simulink model "IEEE_30_Bus_System_with_HVDC"  (R2021a)
settings: Solver=FixedStepDiscrete  StartTime=0.0  StopTime=15  FixedStep=Tss  RelTol=1e-3
InitFcn:
  | Tss=5e-5
  | 
  | Pnom = 20e6
  | Vdc = 40e3
  | 
  | Vbreak_on = Vdc + Vdc*150/800
  | Vbreak_off = Vdc
  | break_status_time = 1.0
  | 
  | Rbrk =  Vdc*Vdc/(1.0*Pnom)
  | 
  | Vg1rms = 33e3*1.0118
  | Lg1 = 20e-6
  | Rg1 = 10e-3
  | f1 = 60.0
  | m_f=27
  | fsw = 10000.0
  | Ilpp = 0.1*Pnom/Vg1rms
  | a = 10.0
  | 
  | ffast = 1.0*fsw
  | Tfast = 1.0/ffast
  | 
  | Rdc = Vdc*Vdc/Pnom
  | 
  | R1 = Vg1rms*Vg1rms / (500*Pnom) / 3.0
  | %L1 = 3.0*1.41*Vg1rms / (2*Vdc) * ((2.0/3.0*Vdc - 1.41*Vg1rms) / (Ilpp*fsw))
  | L1=8e-3
  | %Cf1 = (a+1)/(4*pi*pi*fsw*fsw*Lg1)
  | Cf1=4e-6
  | %C_dc = 100e-10*Pnom
  | C_dc=0.02
  | %R_dump = 1.0/(20.0*pi*f1*Cf1)*10000.0/Pnom
  | R_dump=20
  | 
  | p = -0.135*10.0
  | i = -0.004/2.0
  | 
  | Kp_i = 2*L1*fsw*p / Vdc / 2.0
  | Ki_i = 2*L1*fsw*i / Vdc / 2.0
  | 
  | Tsw = 1/fsw
  | 
  | Vg2rms = 33e3*1.0571
  | Lg2 = 20e-6
  | Rg2 = 10e-3
  | f2 = 60.0
  | fsw2 = 10000.0
  | Il2pp = 0.1*Pnom/Vg2rms
  | a2 = 10.0
  | 
  | R2 = Vg2rms*Vg2rms / (500*Pnom) / 3.0
  | %L2 = 3.0*1.41*Vg2rms / (2*Vdc) * ((2.0/3.0*Vdc - 1.41*Vg2rms) / (Il2pp*fsw2))
  | L2=20e-3
  | %Cf2 = (a2+1)/(4*pi*pi*fsw2*fsw2*Lg2)
  | Cf2=9e-6
  | 
  | %R_dump2 = 1.0/(20.0*pi*f2*Cf2)*10000.0/Pnom
  | R_dump2=20
  | 
  | Tsw2 = 1/fsw2
  | Tslow = 1e-3
  | 
  | p_v = 0.2403
  | i_v = 0.0549
  | 
  | Kp_v = 4*p_v / (1.5*Vg2rms*1.41*Tslow)
  | Ki_v = 4*i_v / (1.5*Vg2rms*1.41*Tslow)
  | 
  | Imax = Pnom/Vg2rms/3.0 * 1.41 * 2.0
undefined symbols (not defined in the file): Angle, DiscIntNeverNeededParam, Magnitude, V_890, Vnom1
libraries: spsThreePhasePISectionLineLib x37, spsThreePhaseVIMeasurementLib x32, spsLoadFlowBusLib x30, spsSeriesRLCBranchLib x27, spsThreePhaseSeriesRLCLoadLib x23, spsVoltageMeasurementLib x17, spsCurrentMeasurementLib x15, spsThreePhaseSourceLib x7, pid_lib x7, spsabctodq0Lib x6, spsFirstOrderFilterLib x4, eeGeneralControl x4
(part 1 of 2)
settings Model: SimulationMode=accelerator  Creator=liyifu  LastModifiedBy=l4729
settings SolverCC: AlgebraicLoopSolver=TrustRegion
settings DataIOCC: ReturnWorkspaceOutputs=off
settings DebuggingCC: UnconnectedInputMsg=none  UnconnectedOutputMsg=none  UnconnectedLineMsg=none  SFMachineParentedDataDiag=warning  ArithmeticOperatorsInVariantConditions=warning
settings SFSimCC: SimUseLocalCustomCode=off  CustomCodeUndefinedFunction=UseInterfaceOnly
settings RTWCC: RTWUseLocalCustomCode=off

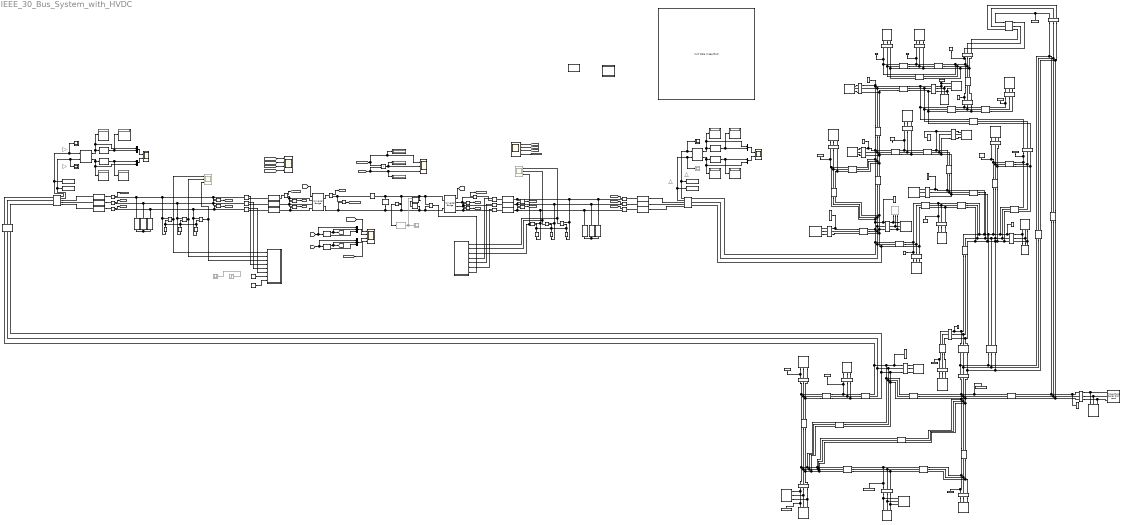
== system IEEE_30_Bus_System_with_HVDC ==
  note: IEEE 30 Node Test Feeder
  14 : spsThreePhaseVIMeasurementLib/Three-Phase V-I Measurement  VoltageMeasurement=phase-to-ground  SetLabelV=on  LabelV=Vabc_14  Vpu=on  VpuLL=off  CurrentMeasurement=yes  SetLabelI=on  LabelI=Iabc_14  Ipu=on  Pbase=100e6  Vbase=33e3  OutputType=Magnitude-Angle  PhasorSimulation=off  PSBequivalent=0
  15 : spsThreePhaseVIMeasurementLib/Three-Phase V-I Measurement  VoltageMeasurement=phase-to-ground  SetLabelV=on  LabelV=Vabc_15  Vpu=on  VpuLL=off  CurrentMeasurement=yes  SetLabelI=on  LabelI=Iabc_15  Ipu=on  Pbase=100e6  Vbase=33e3  OutputType=Magnitude-Angle  PhasorSimulation=off  PSBequivalent=0
  16 : spsThreePhaseVIMeasurementLib/Three-Phase V-I Measurement  VoltageMeasurement=phase-to-ground  SetLabelV=on  LabelV=Vabc_16  Vpu=on  VpuLL=off  CurrentMeasurement=yes  SetLabelI=on  LabelI=Iabc_16  Ipu=on  Pbase=100e6  Vbase=33e3  OutputType=Magnitude-Angle  PhasorSimulation=off  PSBequivalent=0
  17 : spsThreePhaseVIMeasurementLib/Three-Phase V-I Measurement  VoltageMeasurement=phase-to-ground  SetLabelV=on  LabelV=Vabc_17  Vpu=on  VpuLL=off  CurrentMeasurement=yes  SetLabelI=on  LabelI=Iabc_17  Ipu=on  Pbase=100e6  Vbase=33e3  OutputType=Magnitude-Angle  PhasorSimulation=off  PSBequivalent=0
  18 : spsThreePhaseVIMeasurementLib/Three-Phase V-I Measurement  VoltageMeasurement=phase-to-ground  SetLabelV=on  LabelV=Vabc_18  Vpu=on  VpuLL=off  CurrentMeasurement=yes  SetLabelI=on  LabelI=Iabc_18  Ipu=on  Pbase=100e6  Vbase=33e3  OutputType=Magnitude-Angle  PhasorSimulation=off  PSBequivalent=0
  19 : spsThreePhaseVIMeasurementLib/Three-Phase V-I Measurement  VoltageMeasurement=phase-to-ground  SetLabelV=on  LabelV=Vabc_19  Vpu=on  VpuLL=off  CurrentMeasurement=yes  SetLabelI=on  LabelI=Iabc_19  Ipu=on  Pbase=100e6  Vbase=33e3  OutputType=Magnitude-Angle  PhasorSimulation=off  PSBequivalent=0
  20 : spsThreePhaseVIMeasurementLib/Three-Phase V-I Measurement  VoltageMeasurement=phase-to-ground  SetLabelV=on  LabelV=Vabc_20  Vpu=on  VpuLL=off  CurrentMeasurement=yes  SetLabelI=on  LabelI=Iabc_20  Ipu=on  Pbase=100e6  Vbase=33e3  OutputType=Magnitude-Angle  PhasorSimulation=off  PSBequivalent=0
  21 : spsThreePhaseVIMeasurementLib/Three-Phase V-I Measurement  VoltageMeasurement=phase-to-ground  SetLabelV=on  LabelV=Vabc_21  Vpu=on  VpuLL=off  CurrentMeasurement=yes  SetLabelI=on  LabelI=Iabc_21  Ipu=on  Pbase=100e6  Vbase=33e3  OutputType=Magnitude-Angle  PhasorSimulation=off  PSBequivalent=0
  22 : spsThreePhaseVIMeasurementLib/Three-Phase V-I Measurement  VoltageMeasurement=phase-to-ground  SetLabelV=on  LabelV=Vabc_22  Vpu=on  VpuLL=off  CurrentMeasurement=yes  SetLabelI=on  LabelI=Iabc_22  Ipu=on  Pbase=100e6  Vbase=33e3  OutputType=Magnitude-Angle  PhasorSimulation=off  PSBequivalent=0
  23 : spsThreePhaseVIMeasurementLib/Three-Phase V-I Measurement  VoltageMeasurement=phase-to-ground  SetLabelV=on  LabelV=Vabc_23  Vpu=on  VpuLL=off  CurrentMeasurement=yes  SetLabelI=on  LabelI=Iabc_23  Ipu=on  Pbase=100e6  Vbase=33e3  OutputType=Magnitude-Angle  PhasorSimulation=off  PSBequivalent=0
  24 : spsThreePhaseVIMeasurementLib/Three-Phase V-I Measurement  VoltageMeasurement=phase-to-ground  SetLabelV=on  LabelV=Vabc_24  Vpu=on  VpuLL=off  CurrentMeasurement=yes  SetLabelI=on  LabelI=Iabc_24  Ipu=on  Pbase=100e6  Vbase=33e3  OutputType=Magnitude-Angle  PhasorSimulation=off  PSBequivalent=0
  25 : spsThreePhaseVIMeasurementLib/Three-Phase V-I Measurement  VoltageMeasurement=phase-to-ground  SetLabelV=on  LabelV=Vabc_25  Vpu=on  VpuLL=off  CurrentMeasurement=yes  SetLabelI=on  LabelI=Iabc_25  Ipu=on  Pbase=100e6  Vbase=33e3  OutputType=Magnitude-Angle  PhasorSimulation=off  PSBequivalent=0
  26 : spsThreePhaseVIMeasurementLib/Three-Phase V-I Measurement  VoltageMeasurement=phase-to-ground  SetLabelV=on  LabelV=Vabc_26  Vpu=on  VpuLL=off  CurrentMeasurement=yes  SetLabelI=on  LabelI=Iabc_26  Ipu=on  Pbase=100e6  Vbase=33e3  OutputType=Magnitude-Angle  PhasorSimulation=off  PSBequivalent=0
  29 : spsThreePhaseVIMeasurementLib/Three-Phase V-I Measurement  VoltageMeasurement=phase-to-ground  SetLabelV=on  LabelV=Vabc_29  Vpu=on  VpuLL=off  CurrentMeasurement=yes  SetLabelI=on  LabelI=Iabc_29  Ipu=on  Pbase=100e6  Vbase=33e3  OutputType=Magnitude-Angle  PhasorSimulation=off  PSBequivalent=0
  30 : spsThreePhaseVIMeasurementLib/Three-Phase V-I Measurement  VoltageMeasurement=phase-to-ground  SetLabelV=on  LabelV=Vabc_30  Vpu=on  VpuLL=off  CurrentMeasurement=yes  SetLabelI=on  LabelI=Iabc_30  Ipu=on  Pbase=100e6  Vbase=33e3  OutputType=Magnitude-Angle  PhasorSimulation=off  PSBequivalent=0
  Blaine : spsThreePhaseVIMeasurementLib/Three-Phase V-I Measurement  VoltageMeasurement=phase-to-ground  SetLabelV=on  LabelV=Vabc_7  Vpu=on  VpuLL=off  CurrentMeasurement=yes  SetLabelI=on  LabelI=Iabc_7  Ipu=on  Pbase=100e6  Vbase=132e3  OutputType=Magnitude-Angle  PhasorSimulation=off  PSBequivalent=0
  Break control1 : Subsystem  Commented=on
  Breaker1 : spsBreakerLib/Breaker  InitialState=0  SwitchingTimes="[1/60  5/60]"  External=on  BreakerResistance=0.01  SnubberResistance=1e6  SnubberCapacitance=inf  Measurements=None  MoreParameters=on  NoBreakLoop=off
      settings: SourceProductBaseCode=PS
  Claytor : spsThreePhaseVIMeasurementLib/Three-Phase V-I Measurement  VoltageMeasurement=phase-to-ground  SetLabelV=on  LabelV=Vabc_2  Vpu=on  VpuLL=off  CurrentMeasurement=yes  SetLabelI=on  LabelI=Iabc_2  Ipu=on  Pbase=100e6  Vbase=132e3  OutputType=Magnitude-Angle  PhasorSimulation=off  PSBequivalent=0
  Cloverdl : spsThreePhaseVIMeasurementLib/Three-Phase V-I Measurement  VoltageMeasurement=phase-to-ground  SetLabelV=on  LabelV=Vabc_27  Vpu=on  VpuLL=off  CurrentMeasurement=yes  SetLabelI=on  LabelI=Iabc_27  Ipu=on  Pbase=100e6  Vbase=33e3  OutputType=Magnitude-Angle  PhasorSimulation=off  PSBequivalent=0
  Cloverdl1 : spsThreePhaseVIMeasurementLib/Three-Phase V-I Measurement  VoltageMeasurement=phase-to-ground  SetLabelV=on  LabelV=Vabc_28  Vpu=on  VpuLL=off  CurrentMeasurement=yes  SetLabelI=on  LabelI=Iabc_28  Ipu=on  Pbase=100e6  Vbase=132e3  OutputType=Magnitude-Angle  PhasorSimulation=off  PSBequivalent=0
  Constant3 : Constant  Value=5e6
  Constant4 : Constant  Value=1e6
  Current Measurement{1..15} (15 alike) : spsCurrentMeasurementLib/Current Measurement  PhasorSimulation=off  OutputType=Complex  PSBequivalent=0
  Display{1..2,6..8,13..18} (11 alike) : Display
  Equivalent Gen : spsThreePhaseSourceLib/Three-Phase Source  Commented=on  InternalConnection=Yg  VoltagePhases=off  Voltage=(33000)*1.04012  PhaseAngle=92.4376  Voltage_phases=[33 33 33]*1e3/sqrt(3)  PhaseAngles_phases=[0 -120 +120]  Frequency=60  NonIdealSource=on  SpecifyImpedance=off  Resistance=10  Inductance=0.15  ShortCircuitLevel=Apparent_power_gen1  BaseVoltage=33e3  XRratio=8  BusType=PQ  Pref=1000000  Qref=0  Prefabc=[10e3, 10e3, 10e3]  Qrefabc=[0, 0, 0]  Qmin=-Inf  Qmax=Inf
  Fieldale : spsThreePhaseVIMeasurementLib/Three-Phase V-I Measurement  VoltageMeasurement=phase-to-ground  SetLabelV=on  LabelV=Vabc_5  Vpu=on  VpuLL=off  CurrentMeasurement=yes  SetLabelI=on  LabelI=Iabc_5  Ipu=on  Pbase=100e6  Vbase=132e3  OutputType=Magnitude-Angle  PhasorSimulation=off  PSBequivalent=0
  Gain4 : Gain  Commented=on  Gain=33e3*sqrt(2)/sqrt(3)
  Gain5 : Gain  Commented=on  Gain=100e6/33e3*sqrt(2)/sqrt(3)
  Gain6 : Gain  Commented=on  Gain=33e3*sqrt(2)/sqrt(3)
  Gain7 : Gain  Commented=on  Gain=100e6/33e3*sqrt(2)/sqrt(3)
  Gen1 : spsThreePhaseSourceLib/Three-Phase Source  InternalConnection=Yg  VoltagePhases=off  Voltage=(132000)*1.37988  PhaseAngle=133.6021  Voltage_phases=[132 132 132]*1e3/sqrt(3)  PhaseAngles_phases=[0 -120 +120]  Frequency=60  NonIdealSource=on  SpecifyImpedance=off  Resistance=10  Inductance=0.15  ShortCircuitLevel=Apparent_power_gen1  BaseVoltage=132e3  XRratio=8  BusType=swing  Pref=2.6095  Qref=-0.1679  Prefabc=[10e3, 10e3, 10e3]  Qrefabc=[0, 0, 0]  Qmin=-Inf  Qmax=Inf
  Gen2 : spsThreePhaseSourceLib/Three-Phase Source  InternalConnection=Yg  VoltagePhases=off  Voltage=(132000)*1.17992  PhaseAngle=98.3264  Voltage_phases=[132 132 132]*1e3/sqrt(3)  PhaseAngles_phases=[0 -120 +120]  Frequency=60  NonIdealSource=on  SpecifyImpedance=off  Resistance=10  Inductance=0.15  ShortCircuitLevel=Apparent_power_gen1  BaseVoltage=132e3  XRratio=8  BusType=PV  Pref=40000000  Qref=0.5  Prefabc=[10e3, 10e3, 10e3]  Qrefabc=[0, 0, 0]  Qmin=-Inf  Qmax=Inf
  Gen3 : spsThreePhaseSourceLib/Three-Phase Source  InternalConnection=Yg  VoltagePhases=off  Voltage=(132000)*1.11434  PhaseAngle=83.6097  Voltage_phases=[132 132 132]*1e3/sqrt(3)  PhaseAngles_phases=[0 -120 +120]  Frequency=60  NonIdealSource=on  SpecifyImpedance=off  Resistance=10  Inductance=0.15  ShortCircuitLevel=Apparent_power_gen1  BaseVoltage=132e3  XRratio=8  BusType=PV  Pref=0  Qref=0.3685  Prefabc=[10e3, 10e3, 10e3]  Qrefabc=[0, 0, 0]  Qmin=-Inf  Qmax=Inf
  Gen4 : spsThreePhaseSourceLib/Three-Phase Source  InternalConnection=Yg  VoltagePhases=off  Voltage=(132000)*1.0549  PhaseAngle=86.5606  Voltage_phases=[132 132 132]*1e3/sqrt(3)  PhaseAngles_phases=[0 -120 +120]  Frequency=60  NonIdealSource=on  SpecifyImpedance=off  Resistance=10  Inductance=0.15  ShortCircuitLevel=Apparent_power_gen1  BaseVoltage=132e3  XRratio=8  BusType=PV  Pref=0  Qref=0.3714  Prefabc=[10e3, 10e3, 10e3]  Qrefabc=[0, 0, 0]  Qmin=-Inf  Qmax=Inf
  Gen5 : spsThreePhaseSourceLib/Three-Phase Source  InternalConnection=Yg  VoltagePhases=off  Voltage=(33000)*2.66924  PhaseAngle=81.613  Voltage_phases=[33 33 33]*1e3/sqrt(3)  PhaseAngles_phases=[0 -120 +120]  Frequency=60  NonIdealSource=on  SpecifyImpedance=off  Resistance=10  Inductance=0.15  ShortCircuitLevel=Apparent_power_gen1  BaseVoltage=33e3  XRratio=8  BusType=PV  Pref=0  Qref=0.1617  Prefabc=[10e3, 10e3, 10e3]  Qrefabc=[0, 0, 0]  Qmin=-Inf  Qmax=Inf
  Gen6 : spsThreePhaseSourceLib/Three-Phase Source  InternalConnection=Yg  VoltagePhases=off  Voltage=(33000)*2.72717  PhaseAngle=83.0417  Voltage_phases=[33 33 33]*1e3/sqrt(3)  PhaseAngles_phases=[0 -120 +120]  Frequency=60  NonIdealSource=on  SpecifyImpedance=off  Resistance=10  Inductance=0.15  ShortCircuitLevel=Apparent_power_gen1  BaseVoltage=33e3  XRratio=8  BusType=PV  Pref=0  Qref=0.1062  Prefabc=[10e3, 10e3, 10e3]  Qrefabc=[0, 0, 0]  Qmin=-Inf  Qmax=Inf
  Glen Lyn : spsThreePhaseVIMeasurementLib/Three-Phase V-I Measurement  VoltageMeasurement=phase-to-ground  SetLabelV=on  LabelV=Vabc_1  Vpu=on  VpuLL=off  CurrentMeasurement=yes  SetLabelI=on  LabelI=Iabc_1  Ipu=on  Pbase=100e6  Vbase=132e3  OutputType=Magnitude-Angle  PhasorSimulation=off  PSBequivalent=0
  Hancock : spsThreePhaseVIMeasurementLib/Three-Phase V-I Measurement  VoltageMeasurement=phase-to-ground  SetLabelV=on  LabelV=Vabc_4  Vpu=on  VpuLL=off  CurrentMeasurement=yes  SetLabelI=on  LabelI=Iabc_4  Ipu=on  Pbase=100e6  Vbase=132e3  OutputType=Magnitude-Angle  PhasorSimulation=off  PSBequivalent=0
  Hancock1 : spsThreePhaseVIMeasurementLib/Three-Phase V-I Measurement  VoltageMeasurement=phase-to-ground  SetLabelV=on  LabelV=Vabc_12  Vpu=on  VpuLL=off  CurrentMeasurement=yes  SetLabelI=on  LabelI=Iabc_12  Ipu=on  Pbase=100e6  Vbase=33e3  OutputType=Magnitude-Angle  PhasorSimulation=off  PSBequivalent=0
  Hancock2 : spsThreePhaseVIMeasurementLib/Three-Phase V-I Measurement  VoltageMeasurement=phase-to-ground  SetLabelV=on  LabelV=Vabc_13  Vpu=on  VpuLL=off  CurrentMeasurement=yes  SetLabelI=on  LabelI=Iabc_13  Ipu=on  Pbase=100e6  Vbase=33e3  OutputType=Magnitude-Angle  PhasorSimulation=off  PSBequivalent=0
  Inverter Control : Subsystem
  Kumis : spsThreePhaseVIMeasurementLib/Three-Phase V-I Measurement  VoltageMeasurement=phase-to-ground  SetLabelV=on  LabelV=Vabc_3  Vpu=on  VpuLL=off  CurrentMeasurement=yes  SetLabelI=on  LabelI=Iabc_3  Ipu=on  Pbase=100e6  Vbase=132e3  OutputType=Magnitude-Angle  PhasorSimulation=off  PSBequivalent=0
  L1-2 : spsThreePhasePISectionLineLib/Three-Phase PI Section Line  LConnTagsString=a|b|c  RConnTagsString=A|B|C  Length=1  Frequency=60  Resistances=[0.0192 0.048]*174.24  Inductances=[1.5252e-4 3.8131e-4]*174.24  Capacitances=[1.4006e-4 1.4006e-4]/174.24
  L1-3 : spsThreePhasePISectionLineLib/Three-Phase PI Section Line  LConnTagsString=a|b|c  RConnTagsString=A|B|C  Length=1  Frequency=60  Resistances=[0.0452 0.113]*174.24  Inductances=[4.3821e-4 1.0955e-4]*174.24  Capacitances=[1.0823e-4 1.0823e-4]/174.24
  L10-17 : spsThreePhasePISectionLineLib/Three-Phase PI Section Line  LConnTagsString=a|b|c  RConnTagsString=A|B|C  Length=1  Frequency=60  Resistances=[0.0324 0.081]*10.89  Inductances=[2.2414e-4 5.6036e-4]*10.89  Capacitances=[1e-6 1e-6]/10.89
  L10-20 : spsThreePhasePISectionLineLib/Three-Phase PI Section Line  LConnTagsString=a|b|c  RConnTagsString=A|B|C  Length=1  Frequency=60  Resistances=[0.0936 0.234]*10.89  Inductances=[5.5439e-4 1.3860e-3]*10.89  Capacitances=[1e-6 1e-6]/10.89
  L10-21 : spsThreePhasePISectionLineLib/Three-Phase PI Section Line  LConnTagsString=a|b|c  RConnTagsString=A|B|C  Length=1  Frequency=60  Resistances=[0.0348 0.087]*10.89  Inductances=[1.9868e-4 4.9670e-4]*10.89  Capacitances=[1e-6 1e-6]/10.89
  L10-22 : spsThreePhasePISectionLineLib/Three-Phase PI Section Line  LConnTagsString=a|b|c  RConnTagsString=A|B|C  Length=1  Frequency=60  Resistances=[0.0727 0.18175]*10.89  Inductances=[3.9762e-4 9.9406e-4]*10.89  Capacitances=[1e-6 1e-6]/10.89
  L12-13 : spsThreePhasePISectionLineLib/Three-Phase PI Section Line  LConnTagsString=a|b|c  RConnTagsString=A|B|C  Length=1  Frequency=60  Resistances=[0 0]*10.89  Inductances=[3.7136e-4 9.2840e-4]*10.89  Capacitances=[1e-6 1e-6]/10.89
  L12-14 : spsThreePhasePISectionLineLib/Three-Phase PI Section Line  LConnTagsString=a|b|c  RConnTagsString=A|B|C  Length=1  Frequency=60  Resistances=[0.1231 0.30775]*10.89  Inductances=[6.7880e-4 1.6970e-3]*10.89  Capacitances=[1e-6 1e-6]/10.89
  L12-15 : spsThreePhasePISectionLineLib/Three-Phase PI Section Line  LConnTagsString=a|b|c  RConnTagsString=A|B|C  Length=1  Frequency=60  Resistances=[0.0662 0.1655]*10.89  Inductances=[3.4590e-4 8.6474e-4]*10.89  Capacitances=[1e-6 1e-6]/10.89
  L12-16 : spsThreePhasePISectionLineLib/Three-Phase PI Section Line  LConnTagsString=a|b|c  RConnTagsString=A|B|C  Length=1  Frequency=60  Resistances=[0.0945 0.23625]*10.89  Inductances=[5.2707e-4 1.3177e-3]*10.89  Capacitances=[1e-6 1e-6]/10.89
  L14-15 : spsThreePhasePISectionLineLib/Three-Phase PI Section Line  LConnTagsString=a|b|c  RConnTagsString=A|B|C  Length=1  Frequency=60  Resistances=[0.221 0.5525]*10.89  Inductances=[5.2972e-4 1.3243e-3]*10.89  Capacitances=[1e-6 1e-6]/10.89
  L15-18 : spsThreePhasePISectionLineLib/Three-Phase PI Section Line  LConnTagsString=a|b|c  RConnTagsString=A|B|C  Length=1  Frequency=60  Resistances=[0.1073 0.26825]*10.89  Inductances=[5.7959e-4 1.4490e-3]*10.89  Capacitances=[1e-6 1e-6]/10.89
  L15-23 : spsThreePhasePISectionLineLib/Three-Phase PI Section Line  LConnTagsString=a|b|c  RConnTagsString=A|B|C  Length=1  Frequency=60  Resistances=[0.1 0.25]*10.89  Inductances=[5.3582e-4 1.3396e-3]*10.89  Capacitances=[1e-6 1e-6]/10.89
  L16-17 : spsThreePhasePISectionLineLib/Three-Phase PI Section Line  LConnTagsString=a|b|c  RConnTagsString=A|B|C  Length=1  Frequency=60  Resistances=[0.0524 0.131]*10.89  Inductances=[5.1009e-4 1.2752e-3]*10.89  Capacitances=[1e-6 1e-6]/10.89
  L18-19 : spsThreePhasePISectionLineLib/Three-Phase PI Section Line  LConnTagsString=a|b|c  RConnTagsString=A|B|C  Length=1  Frequency=60  Resistances=[0.0639 0.15975]*10.89  Inductances=[3.4271e-4 8.5678e-4]*10.89  Capacitances=[1e-6 1e-6]/10.89
  L19-20 : spsThreePhasePISectionLineLib/Three-Phase PI Section Line  LConnTagsString=a|b|c  RConnTagsString=A|B|C  Length=1  Frequency=60  Resistances=[0.034 0.085]*10.89  Inductances=[1.8038e-4 4.5094e-4]*10.89  Capacitances=[1e-6 1e-6]/10.89
  L2-4 : spsThreePhasePISectionLineLib/Three-Phase PI Section Line  LConnTagsString=a|b|c  RConnTagsString=A|B|C  Length=1  Frequency=60  Resistances=[0.057 0.1425]*174.24  Inductances=[4.6075e-4 1.1519e-3]*174.24  Capacitances=[9.7615e-5 9.7615e-5]/174.24
  L2-5 : spsThreePhasePISectionLineLib/Three-Phase PI Section Line  LConnTagsString=a|b|c  RConnTagsString=A|B|C  Length=1  Frequency=60  Resistances=[0.0472 0.118]*174.24  Inductances=[5.2601e-4 1.3150e-3]*174.24  Capacitances=[1.1088e-4 1.1088e-4]/174.24
  L2-6 : spsThreePhasePISectionLineLib/Three-Phase PI Section Line  LConnTagsString=a|b|c  RConnTagsString=A|B|C  Length=1  Frequency=60  Resistances=[0.0581 0.14525]*174.24  Inductances=[4.6765e-4 1.1691e-3]*174.24  Capacitances=[9.9206e-5 9.9206e-5]/174.24
  L21-22 : spsThreePhasePISectionLineLib/Three-Phase PI Section Line  LConnTagsString=a|b|c  RConnTagsString=A|B|C  Length=1  Frequency=60  Resistances=[0.0116 0.029]*10.89  Inductances=[6.2601e-5 1.5650e-4]*10.89  Capacitances=[1e-6 1e-6]/10.89
  L22-24 : spsThreePhasePISectionLineLib/Three-Phase PI Section Line  LConnTagsString=a|b|c  RConnTagsString=A|B|C  Length=1  Frequency=60  Resistances=[0.115 0.2875]*10.89  Inductances=[4.7481e-4 1.1870e-3]*10.89  Capacitances=[1e-6 1e-6]/10.89
  L23-24 : spsThreePhasePISectionLineLib/Three-Phase PI Section Line  LConnTagsString=a|b|c  RConnTagsString=A|B|C  Length=1  Frequency=60  Resistances=[0.132 0.33]*10.89  Inductances=[7.1620e-4 1.7905e-3]*10.89  Capacitances=[1e-6 1e-6]/10.89
  L24-25 : spsThreePhasePISectionLineLib/Three-Phase PI Section Line  LConnTagsString=a|b|c  RConnTagsString=A|B|C  Length=1  Frequency=60  Resistances=[0.1885 0.47125]*10.89  Inductances=[8.7323e-4 2.1831e-3]*10.89  Capacitances=[1e-6 1e-6]/10.89
  L25-26 : spsThreePhasePISectionLineLib/Three-Phase PI Section Line  LConnTagsString=a|b|c  RConnTagsString=A|B|C  Length=1  Frequency=60  Resistances=[0.2544 0.636]*10.89  Inductances=[1.008e-3 2.5200e-3]*10.89  Capacitances=[1e-6 1e-6]/10.89
  L25-27 : spsThreePhasePISectionLineLib/Three-Phase PI Section Line  LConnTagsString=a|b|c  RConnTagsString=A|B|C  Length=1  Frequency=60  Resistances=[0.1093 0.27325]*10.89  Inductances=[5.5360e-4 1.3840e-3]*10.89  Capacitances=[1e-6 1e-6]/10.89
  L27-29 : spsThreePhasePISectionLineLib/Three-Phase PI Section Line  LConnTagsString=a|b|c  RConnTagsString=A|B|C  Length=1  Frequency=60  Resistances=[0.2198 0.5495]*10.89  Inductances=[1.1016e-3 2.7540e-3]*10.89  Capacitances=[1e-6 1e-6]/10.89
  L27-30 : spsThreePhasePISectionLineLib/Three-Phase PI Section Line  LConnTagsString=a|b|c  RConnTagsString=A|B|C  Length=1  Frequency=60  Resistances=[0.3202 0.8005]*10.89  Inductances=[1.5987e-3 3.9968e-3]*10.89  Capacitances=[1e-6 1e-6]/10.89
  L29-30 : spsThreePhasePISectionLineLib/Three-Phase PI Section Line  LConnTagsString=a|b|c  RConnTagsString=A|B|C  Length=1  Frequency=60  Resistances=[0.2399 0.59975]*10.89  Inductances=[1.2024e-3 3.0060e-3]*10.89  Capacitances=[1e-6 1e-6]/10.89
  L3-4 : spsThreePhasePISectionLineLib/Three-Phase PI Section Line  LConnTagsString=a|b|c  RConnTagsString=A|B|C  Length=1  Frequency=60  Resistances=[0.0132 0.033]*174.24  Inductances=[1.0053e-4 2.5133e-4]*174.24  Capacitances=[2.2282e-5 2.2282e-5]/174.24
  L4-6 : spsThreePhasePISectionLineLib/Three-Phase PI Section Line  LConnTagsString=a|b|c  RConnTagsString=A|B|C  Length=1  Frequency=60  Resistances=[0.0119 0.02975]*174.24  Inductances=[1.0982e-4 2.7452e-4]*174.24  Capacitances=[2.3873e-5 2.3873e-5]/174.24
  L5-7 : spsThreePhasePISectionLineLib/Three-Phase PI Section Line  LConnTagsString=a|b|c  RConnTagsString=A|B|C  Length=1  Frequency=60  Resistances=[0.046 0.115]*174.24  Inductances=[3.0770e-4 7.6925e-4]*174.24  Capacitances=[5.4113e-5 5.4113e-5]/174.24
  L6-28 : spsThreePhasePISectionLineLib/Three-Phase PI Section Line  LConnTagsString=a|b|c  RConnTagsString=A|B|C  Length=1  Frequency=60  Resistances=[0.0169 0.04225]*174.24  Inductances=[1.5889e-4 3.9722e-4]*174.24  Capacitances=[3.4484e-5 3.4484e-5]/174.24
  L6-7 : spsThreePhasePISectionLineLib/Three-Phase PI Section Line  LConnTagsString=a|b|c  RConnTagsString=A|B|C  Length=1  Frequency=60  Resistances=[0.0267 0.06675]*174.24  Inductances=[2.1751e-4 5.4378e-4]*174.24  Capacitances=[4.5094e-5 4.5094e-5]/174.24
  L6-8 : spsThreePhasePISectionLineLib/Three-Phase PI Section Line  LConnTagsString=a|b|c  RConnTagsString=A|B|C  Length=1  Frequency=60  Resistances=[0.012 0.03]*174.24  Inductances=[1.1141e-4 2.7852e-4]*174.24  Capacitances=[2.3873e-5 2.3873e-5]/174.24
  L8-28 : spsThreePhasePISectionLineLib/Three-Phase PI Section Line  LConnTagsString=a|b|c  RConnTagsString=A|B|C  Length=1  Frequency=60  Resistances=[0.0636 0.159]*174.24  Inductances=[5.3052e-4 1.3263e-3]*174.24  Capacitances=[1.1353e-4 1.1353e-4]/174.24
  L9-10 : spsThreePhasePISectionLineLib/Three-Phase PI Section Line  LConnTagsString=a|b|c  RConnTagsString=A|B|C  Length=1  Frequency=60  Resistances=[0 0]*10.89  Inductances=[2.9178e-4 7.2946e-4]*10.89  Capacitances=[1e-6 1e-6]/10.89
  L9-11 : spsThreePhasePISectionLineLib/Three-Phase PI Section Line  LConnTagsString=a|b|c  RConnTagsString=A|B|C  Length=1  Frequency=60  Resistances=[0 0]*10.89  Inductances=[5.5174e-4 1.3793e-3]*10.89  Capacitances=[1e-6 1e-6]/10.89
  Load Flow Bus1 : spsLoadFlowBusLib/Load Flow Bus  LConnTagsString=a  Phases=single  Connectors=on both sides  ID=BUS5  Vbase=132e3  Vref=1*1.0100  Vangle=84.266  VLF=1.01  VLFb=1  VLFc=1  angleLF=84.56  angleLFb=0  angleLFc=0
      settings: AttributesFormatString=%<ID>  SourceProductBaseCode=PS
  Load Flow Bus10 : spsLoadFlowBusLib/Load Flow Bus  LConnTagsString=a  Phases=single  Connectors=on both sides  ID=BUS25  Vbase=33e3  Vref=1*1.0173  Vangle=82.365  VLF=1.001  VLFb=1  VLFc=1  angleLF=86.72  angleLFb=0  angleLFc=0
      settings: AttributesFormatString=%<ID>  SourceProductBaseCode=PS
  Load Flow Bus11 : spsLoadFlowBusLib/Load Flow Bus  LConnTagsString=a  Phases=single  Connectors=on both sides  ID=BUS29  Vbase=33e3  Vref=1*1.0034  Vangle=81.659  VLF=0.9927  VLFb=1  VLFc=1  angleLF=85.75  angleLFb=0  angleLFc=0
      settings: AttributesFormatString=%<ID>  SourceProductBaseCode=PS
  Load Flow Bus12 : spsLoadFlowBusLib/Load Flow Bus  LConnTagsString=a  Phases=single  Connectors=on both sides  ID=BUS30  Vbase=33e3  Vref=1*0.9919  Vangle=80.776  VLF=0.9811  VLFb=1  VLFc=1  angleLF=84.85  angleLFb=0  angleLFc=0
      settings: AttributesFormatString=%<ID>  SourceProductBaseCode=PS
  Load Flow Bus13 : spsLoadFlowBusLib/Load Flow Bus  LConnTagsString=a  Phases=single  Connectors=on both sides  ID=BUS22  Vbase=33e3  Vref=1*1.0333  Vangle=82.303  VLF=1.007  VLFb=1  VLFc=1  angleLF=87.09  angleLFb=0  angleLFc=0
      settings: AttributesFormatString=%<ID>  SourceProductBaseCode=PS
  Load Flow Bus2 : spsLoadFlowBusLib/Load Flow Bus  LConnTagsString=a  Phases=single  Connectors=on both sides  ID=BUS18  Vbase=33e3  Vref=1*1.0282  Vangle=81.890  VLF=0.9994  VLFb=1  VLFc=1  angleLF=87.02  angleLFb=0  angleLFc=0
      settings: AttributesFormatString=%<ID>  SourceProductBaseCode=PS
  Load Flow Bus28 : spsLoadFlowBusLib/Load Flow Bus  LConnTagsString=a  Phases=single  Connectors=on both sides  ID=BUS1  Vbase=132e3  Vref=1*1.06  Vangle=98.432  VLF=1.06  VLFb=1  VLFc=1  angleLF=98.43  angleLFb=0  angleLFc=0
      settings: AttributesFormatString=%<ID>  SourceProductBaseCode=PS
  Load Flow Bus3 : spsLoadFlowBusLib/Load Flow Bus  LConnTagsString=a  Phases=single  Connectors=on both sides  ID=BUS4  Vbase=132e3  Vref=1*1.0118  Vangle=89.148  VLF=1.027  VLFb=1  VLFc=1  angleLF=89.19  angleLFb=0  angleLFc=0
      settings: AttributesFormatString=%<ID>  SourceProductBaseCode=PS
  Load Flow Bus37 : spsLoadFlowBusLib/Load Flow Bus  LConnTagsString=a  Phases=single  Connectors=on both sides  ID=BUS2  Vbase=132e3  Vref=1*1.0431  Vangle=93.080  VLF=1.043  VLFb=1  VLFc=1  angleLF=93.22  angleLFb=0  angleLFc=0
      settings: AttributesFormatString=%<ID>  SourceProductBaseCode=PS
  Load Flow Bus4 : spsLoadFlowBusLib/Load Flow Bus  LConnTagsString=a  Phases=single  Connectors=on both sides  ID=BUS3  Vbase=132e3  Vref=1*1.0207  Vangle=90.900  VLF=1.033  VLFb=1  VLFc=1  angleLF=90.92  angleLFb=0  angleLFc=0
      settings: AttributesFormatString=%<ID>  SourceProductBaseCode=PS
  Load Flow Bus42 : spsLoadFlowBusLib/Load Flow Bus  LConnTagsString=a  Phases=single  Connectors=on one side  ID=BUS7  Vbase=132e3  Vref=1*1.0024  Vangle=85.566  VLF=1.007  VLFb=1  VLFc=1  angleLF=85.82  angleLFb=0  angleLFc=0
      settings: AttributesFormatString=%<ID>  SourceProductBaseCode=PS
  Load Flow Bus43 : spsLoadFlowBusLib/Load Flow Bus  LConnTagsString=a  Phases=single  Connectors=on both sides  ID=BUS6  Vbase=132e3  Vref=1*1.0103  Vangle=87.367  VLF=1.019  VLFb=1  VLFc=1  angleLF=87.59  angleLFb=0  angleLFc=0
      settings: AttributesFormatString=%<ID>  SourceProductBaseCode=PS
  Load Flow Bus44 : spsLoadFlowBusLib/Load Flow Bus  LConnTagsString=a  Phases=single  Connectors=on both sides  ID=BUS8  Vbase=132e3  Vref=1*1.0100  Vangle=86.618  VLF=1.01  VLFb=1  VLFc=1  angleLF=86.99  angleLFb=0  angleLFc=0
      settings: AttributesFormatString=%<ID>  SourceProductBaseCode=PS
  Load Flow Bus45 : spsLoadFlowBusLib/Load Flow Bus  LConnTagsString=a  Phases=single  Connectors=on one side  ID=BUS28  Vbase=132e3  Vref=1*1.0068  Vangle=86.743  VLF=1.013  VLFb=1  VLFc=1  angleLF=87.03  angleLFb=0  angleLFc=0
      settings: AttributesFormatString=%<ID>  SourceProductBaseCode=PS
  Load Flow Bus46 : spsLoadFlowBusLib/Load Flow Bus  LConnTagsString=a  Phases=single  Connectors=on one side  ID=BUS27  Vbase=33e3  Vref=1*1.0232  Vangle=82.889  VLF=1.013  VLFb=1  VLFc=1  angleLF=87.01  angleLFb=0  angleLFc=0
      settings: AttributesFormatString=%<ID>  SourceProductBaseCode=PS
  Load Flow Bus5 : spsLoadFlowBusLib/Load Flow Bus  LConnTagsString=a  Phases=single  Connectors=on both sides  ID=BUS14  Vbase=33e3  Vref=1*1.0423  Vangle=82.596  VLF=1.013  VLFb=1  VLFc=1  angleLF=88.1  angleLFb=0  angleLFc=0
      settings: AttributesFormatString=%<ID>  SourceProductBaseCode=PS
  Load Flow Bus52 : spsLoadFlowBusLib/Load Flow Bus  LConnTagsString=a  Phases=single  Connectors=on both sides  ID=BUS23  Vbase=33e3  Vref=1*1.0272  Vangle=82.114  VLF=0.9999  VLFb=1  VLFc=1  angleLF=87.22  angleLFb=0  angleLFc=0
      settings: AttributesFormatString=%<ID>  SourceProductBaseCode=PS
  Load Flow Bus53 : spsLoadFlowBusLib/Load Flow Bus  LConnTagsString=a  Phases=single  Connectors=on both sides  ID=BUS9  Vbase=33e3  Vref=1*1.0509  Vangle=84.323  VLF=1.019  VLFb=1  VLFc=1  angleLF=87.59  angleLFb=0  angleLFc=0
      settings: AttributesFormatString=%<ID>  SourceProductBaseCode=PS
  Load Flow Bus54 : spsLoadFlowBusLib/Load Flow Bus  LConnTagsString=a  Phases=single  Connectors=on both sides  ID=BUS10  Vbase=33e3  Vref=1*1.0451  Vangle=82.732  VLF=1.018  VLFb=1  VLFc=1  angleLF=87.53  angleLFb=0  angleLFc=0
      settings: AttributesFormatString=%<ID>  SourceProductBaseCode=PS
  Load Flow Bus55 : spsLoadFlowBusLib/Load Flow Bus  LConnTagsString=a  Phases=single  Connectors=on both sides  ID=BUS17  Vbase=33e3  Vref=1*1.0399  Vangle=82.570  VLF=1.012  VLFb=1  VLFc=1  angleLF=87.51  angleLFb=0  angleLFc=0
      settings: AttributesFormatString=%<ID>  SourceProductBaseCode=PS
  Load Flow Bus56 : spsLoadFlowBusLib/Load Flow Bus  LConnTagsString=a  Phases=single  Connectors=on both sides  ID=BUS16  Vbase=33e3  Vref=1*1.0444  Vangle=82.905  VLF=1.015  VLFb=1  VLFc=1  angleLF=88.17  angleLFb=0  angleLFc=0
      settings: AttributesFormatString=%<ID>  SourceProductBaseCode=PS
  Load Flow Bus57 : spsLoadFlowBusLib/Load Flow Bus  LConnTagsString=a  Phases=single  Connectors=on both sides  ID=BUS12  Vbase=33e3  Vref=1*1.0571  Vangle=83.488  VLF=1.027  VLFb=1  VLFc=1  angleLF=89.15  angleLFb=0  angleLFc=0
      settings: AttributesFormatString=%<ID>  SourceProductBaseCode=PS
  Load Flow Bus58 : spsLoadFlowBusLib/Load Flow Bus  LConnTagsString=a  Phases=single  Connectors=on both sides  ID=BUS13  Vbase=33e3  Vref=1*1.0710  Vangle=83.488  VLF=1.071  VLFb=1  VLFc=1  angleLF=89.15  angleLFb=0  angleLFc=0
      settings: AttributesFormatString=%<ID>  SourceProductBaseCode=PS
  Load Flow Bus6 : spsLoadFlowBusLib/Load Flow Bus  LConnTagsString=a  Phases=single  Connectors=on both sides  ID=BUS21  Vbase=33e3  Vref=1*1.0327  Vangle=82.289  VLF=1.006  VLFb=1  VLFc=1  angleLF=87.07  angleLFb=0  angleLFc=0
      settings: AttributesFormatString=%<ID>  SourceProductBaseCode=PS
  Load Flow Bus62 : spsLoadFlowBusLib/Load Flow Bus  LConnTagsString=a  Phases=single  Connectors=on both sides  ID=BUS20  Vbase=33e3  Vref=1*1.0297  Vangle=81.913  VLF=1.002  VLFb=1  VLFc=1  angleLF=86.85  angleLFb=0  angleLFc=0
      settings: AttributesFormatString=%<ID>  SourceProductBaseCode=PS
  Load Flow Bus63 : spsLoadFlowBusLib/Load Flow Bus  LConnTagsString=a  Phases=single  Connectors=on both sides  ID=BUS11  Vbase=33e3  Vref=1*1.0820  Vangle=84.323  VLF=1.082  VLFb=1  VLFc=1  angleLF=87.59  angleLFb=0  angleLFc=0
      settings: AttributesFormatString=%<ID>  SourceProductBaseCode=PS
  Load Flow Bus64 : spsLoadFlowBusLib/Load Flow Bus  LConnTagsString=a  Phases=single  Connectors=on both sides  ID=BUS15  Vbase=33e3  Vref=1*1.0377  Vangle=82.504  VLF=1.008  VLFb=1  VLFc=1  angleLF=87.88  angleLFb=0  angleLFc=0
      settings: AttributesFormatString=%<ID>  SourceProductBaseCode=PS
  Load Flow Bus7 : spsLoadFlowBusLib/Load Flow Bus  LConnTagsString=a  Phases=single  Connectors=on both sides  ID=BUS19  Vbase=33e3  Vref=1*1.0257  Vangle=81.716  VLF=0.9974  VLFb=1  VLFc=1  angleLF=86.71  angleLFb=0  angleLFc=0
      settings: AttributesFormatString=%<ID>  SourceProductBaseCode=PS
  Load Flow Bus8 : spsLoadFlowBusLib/Load Flow Bus  LConnTagsString=a  Phases=single  Connectors=on both sides  ID=BUS26  Vbase=33e3  Vref=1*0.9997  Vangle=81.945  VLF=0.9835  VLFb=1  VLFc=1  angleLF=86.28  angleLFb=0  angleLFc=0
      settings: AttributesFormatString=%<ID>  SourceProductBaseCode=PS
  Load Flow Bus9 : spsLoadFlowBusLib/Load Flow Bus  LConnTagsString=a  Phases=single  Connectors=on both sides  ID=BUS24  Vbase=33e3  Vref=1*1.0216  Vangle=81.937  VLF=0.9974  VLFb=1  VLFc=1  angleLF=86.7  angleLFb=0  angleLFc=0
      settings: AttributesFormatString=%<ID>  SourceProductBaseCode=PS
  Load10 : spsThreePhaseSeriesRLCLoadLib/Three-Phase Series RLC Load  LConnTagsString=A|B|C  Configuration=Y (grounded)  NominalVoltage=(33000)*1.01845  Vabc=[1e3 1e3 1e3]  Vabcp=V_890*Vnom1  NominalFrequency=60  UnbalancedPower=off  ActivePower=5800000  InductivePower=2000000  CapacitivePower=0  Pabc=[10e3 9e3 11e3]  QLabc=[100 90 110]  QCabc=[100 90 110]  Pabcp=Pa_890  QLabcp=Pp_890  QCabcp=Pn_890  Measurements=None  LoadType=constant PQ
  Load12 : spsThreePhaseSeriesRLCLoadLib/Three-Phase Series RLC Load  LConnTagsString=A|B|C  Configuration=Y (grounded)  NominalVoltage=(33000)*1.02674  Vabc=[1e3 1e3 1e3]  Vabcp=V_890*Vnom1  NominalFrequency=60  UnbalancedPower=off  ActivePower=11.2e6  InductivePower=7.5e6  CapacitivePower=0  Pabc=[10e3 9e3 11e3]  QLabc=[100 90 110]  QCabc=[100 90 110]  Pabcp=Pa_890  QLabcp=Pp_890  QCabcp=Pn_890  Measurements=None  LoadType=constant PQ
  Load14 : spsThreePhaseSeriesRLCLoadLib/Three-Phase Series RLC Load  LConnTagsString=A|B|C  Configuration=Y (grounded)  NominalVoltage=(33000)*1.01262  Vabc=[1e3 1e3 1e3]  Vabcp=V_890*Vnom1  NominalFrequency=60  UnbalancedPower=off  ActivePower=6200000  InductivePower=1600000  CapacitivePower=0  Pabc=[10e3 9e3 11e3]  QLabc=[100 90 110]  QCabc=[100 90 110]  Pabcp=Pa_890  QLabcp=Pp_890  QCabcp=Pn_890  Measurements=None  LoadType=constant PQ
  Load15 : spsThreePhaseSeriesRLCLoadLib/Three-Phase Series RLC Load  LConnTagsString=A|B|C  Configuration=Y (grounded)  NominalVoltage=(33000)*1.00825  Vabc=[1e3 1e3 1e3]  Vabcp=V_890*Vnom1  NominalFrequency=60  UnbalancedPower=off  ActivePower=8200000  InductivePower=2500000  CapacitivePower=0  Pabc=[10e3 9e3 11e3]  QLabc=[100 90 110]  QCabc=[100 90 110]  Pabcp=Pa_890  QLabcp=Pp_890  QCabcp=Pn_890  Measurements=None  LoadType=constant PQ
  Load16 : spsThreePhaseSeriesRLCLoadLib/Three-Phase Series RLC Load  LConnTagsString=A|B|C  Configuration=Y (grounded)  NominalVoltage=(33000)*1.01484  Vabc=[1e3 1e3 1e3]  Vabcp=V_890*Vnom1  NominalFrequency=60  UnbalancedPower=off  ActivePower=3500000  InductivePower=1800000  CapacitivePower=0  Pabc=[10e3 9e3 11e3]  QLabc=[100 90 110]  QCabc=[100 90 110]  Pabcp=Pa_890  QLabcp=Pp_890  QCabcp=Pn_890  Measurements=None  LoadType=constant PQ
  Load17 : spsThreePhaseSeriesRLCLoadLib/Three-Phase Series RLC Load  LConnTagsString=A|B|C  Configuration=Y (grounded)  NominalVoltage=(33000)*1.01238  Vabc=[1e3 1e3 1e3]  Vabcp=V_890*Vnom1  NominalFrequency=60  UnbalancedPower=off  ActivePower=9000000  InductivePower=5800000  CapacitivePower=0  Pabc=[10e3 9e3 11e3]  QLabc=[100 90 110]  QCabc=[100 90 110]  Pabcp=Pa_890  QLabcp=Pp_890  QCabcp=Pn_890  Measurements=None  LoadType=constant PQ
  Load18 : spsThreePhaseSeriesRLCLoadLib/Three-Phase Series RLC Load  LConnTagsString=A|B|C  Configuration=Y (grounded)  NominalVoltage=(33000)*0.999393  Vabc=[1e3 1e3 1e3]  Vabcp=V_890*Vnom1  NominalFrequency=60  UnbalancedPower=off  ActivePower=3200000  InductivePower=900000  CapacitivePower=0  Pabc=[10e3 9e3 11e3]  QLabc=[100 90 110]  QCabc=[100 90 110]  Pabcp=Pa_890  QLabcp=Pp_890  QCabcp=Pn_890  Measurements=None  LoadType=constant PQ
  Load19 : spsThreePhaseSeriesRLCLoadLib/Three-Phase Series RLC Load  LConnTagsString=A|B|C  Configuration=Y (grounded)  NominalVoltage=(33000)*0.997368  Vabc=[1e3 1e3 1e3]  Vabcp=V_890*Vnom1  NominalFrequency=60  UnbalancedPower=off  ActivePower=9500000  InductivePower=3400000  CapacitivePower=0  Pabc=[10e3 9e3 11e3]  QLabc=[100 90 110]  QCabc=[100 90 110]  Pabcp=Pa_890  QLabcp=Pp_890  QCabcp=Pn_890  Measurements=None  LoadType=constant PQ
  Load2 : spsThreePhaseSeriesRLCLoadLib/Three-Phase Series RLC Load  LConnTagsString=A|B|C  Configuration=Y (grounded)  NominalVoltage=(132000)*1.0431  Vabc=[1e3 1e3 1e3]  Vabcp=V_890*Vnom1  NominalFrequency=60  UnbalancedPower=off  ActivePower=21700000  InductivePower=12700000  CapacitivePower=0  Pabc=[10e3 9e3 11e3]  QLabc=[100 90 110]  QCabc=[100 90 110]  Pabcp=Pa_890  QLabcp=Pp_890  QCabcp=Pn_890  Measurements=None  LoadType=constant PQ
  Load20 : spsThreePhaseSeriesRLCLoadLib/Three-Phase Series RLC Load  LConnTagsString=A|B|C  Configuration=Y (grounded)  NominalVoltage=(33000)*1.00183  Vabc=[1e3 1e3 1e3]  Vabcp=V_890*Vnom1  NominalFrequency=60  UnbalancedPower=off  ActivePower=2200000  InductivePower=700000  CapacitivePower=0  Pabc=[10e3 9e3 11e3]  QLabc=[100 90 110]  QCabc=[100 90 110]  Pabcp=Pa_890  QLabcp=Pp_890  QCabcp=Pn_890  Measurements=None  LoadType=constant PQ
  Load21 : spsThreePhaseSeriesRLCLoadLib/Three-Phase Series RLC Load  LConnTagsString=A|B|C  Configuration=Y (grounded)  NominalVoltage=(33000)*1.00632  Vabc=[1e3 1e3 1e3]  Vabcp=V_890*Vnom1  NominalFrequency=60  UnbalancedPower=off  ActivePower=17500000  InductivePower=11200000  CapacitivePower=0  Pabc=[10e3 9e3 11e3]  QLabc=[100 90 110]  QCabc=[100 90 110]  Pabcp=Pa_890  QLabcp=Pp_890  QCabcp=Pn_890  Measurements=None  LoadType=constant PQ
  Load23 : spsThreePhaseSeriesRLCLoadLib/Three-Phase Series RLC Load  LConnTagsString=A|B|C  Configuration=Y (grounded)  NominalVoltage=(33000)*0.999907  Vabc=[1e3 1e3 1e3]  Vabcp=V_890*Vnom1  NominalFrequency=60  UnbalancedPower=off  ActivePower=3200000  InductivePower=1600000  CapacitivePower=0  Pabc=[10e3 9e3 11e3]  QLabc=[100 90 110]  QCabc=[100 90 110]  Pabcp=Pa_890  QLabcp=Pp_890  QCabcp=Pn_890  Measurements=None  LoadType=constant PQ
  Load24 : spsThreePhaseSeriesRLCLoadLib/Three-Phase Series RLC Load  LConnTagsString=A|B|C  Configuration=Y (grounded)  NominalVoltage=(33000)*0.997437  Vabc=[1e3 1e3 1e3]  Vabcp=V_890*Vnom1  NominalFrequency=60  UnbalancedPower=off  ActivePower=8700000  InductivePower=6700000  CapacitivePower=0  Pabc=[10e3 9e3 11e3]  QLabc=[100 90 110]  QCabc=[100 90 110]  Pabcp=Pa_890  QLabcp=Pp_890  QCabcp=Pn_890  Measurements=None  LoadType=constant PQ
  Load26 : spsThreePhaseSeriesRLCLoadLib/Three-Phase Series RLC Load  LConnTagsString=A|B|C  Configuration=Y (grounded)  NominalVoltage=(33000)*0.983528  Vabc=[1e3 1e3 1e3]  Vabcp=V_890*Vnom1  NominalFrequency=60  UnbalancedPower=off  ActivePower=3500000  InductivePower=2300000  CapacitivePower=0  Pabc=[10e3 9e3 11e3]  QLabc=[100 90 110]  QCabc=[100 90 110]  Pabcp=Pa_890  QLabcp=Pp_890  QCabcp=Pn_890  Measurements=None  LoadType=constant PQ
  Load29 : spsThreePhaseSeriesRLCLoadLib/Three-Phase Series RLC Load  LConnTagsString=A|B|C  Configuration=Y (grounded)  NominalVoltage=(33000)*0.992663  Vabc=[1e3 1e3 1e3]  Vabcp=V_890*Vnom1  NominalFrequency=60  UnbalancedPower=off  ActivePower=2400000  InductivePower=900000  CapacitivePower=0  Pabc=[10e3 9e3 11e3]  QLabc=[100 90 110]  QCabc=[100 90 110]  Pabcp=Pa_890  QLabcp=Pp_890  QCabcp=Pn_890  Measurements=None  LoadType=constant PQ
  Load3 : spsThreePhaseSeriesRLCLoadLib/Three-Phase Series RLC Load  LConnTagsString=A|B|C  Configuration=Y (grounded)  NominalVoltage=(132000)*1.03274  Vabc=[1e3 1e3 1e3]  Vabcp=V_890*Vnom1  NominalFrequency=60  UnbalancedPower=off  ActivePower=2400000  InductivePower=1200000  CapacitivePower=0  Pabc=[10e3 9e3 11e3]  QLabc=[100 90 110]  QCabc=[100 90 110]  Pabcp=Pa_890  QLabcp=Pp_890  QCabcp=Pn_890  Measurements=None  LoadType=constant PQ
  Load30 : spsThreePhaseSeriesRLCLoadLib/Three-Phase Series RLC Load  LConnTagsString=A|B|C  Configuration=Y (grounded)  NominalVoltage=(33000)*0.981078  Vabc=[1e3 1e3 1e3]  Vabcp=V_890*Vnom1  NominalFrequency=60  UnbalancedPower=off  ActivePower=10600000  InductivePower=1900000  CapacitivePower=0  Pabc=[10e3 9e3 11e3]  QLabc=[100 90 110]  QCabc=[100 90 110]  Pabcp=Pa_890  QLabcp=Pp_890  QCabcp=Pn_890  Measurements=None  LoadType=constant PQ
  Load4 : spsThreePhaseSeriesRLCLoadLib/Three-Phase Series RLC Load  LConnTagsString=A|B|C  Configuration=Y (grounded)  NominalVoltage=(132000)*1.02653  Vabc=[1e3 1e3 1e3]  Vabcp=V_890*Vnom1  NominalFrequency=60  UnbalancedPower=off  ActivePower=7.6e6  InductivePower=1.6e6  CapacitivePower=0  Pabc=[10e3 9e3 11e3]  QLabc=[100 90 110]  QCabc=[100 90 110]  Pabcp=Pa_890  QLabcp=Pp_890  QCabcp=Pn_890  Measurements=None  LoadType=constant PQ
  Load5 : spsThreePhaseSeriesRLCLoadLib/Three-Phase Series RLC Load  LConnTagsString=A|B|C  Configuration=Y (grounded)  NominalVoltage=(132000)*1.01  Vabc=[1e3 1e3 1e3]  Vabcp=V_890*Vnom1  NominalFrequency=60  UnbalancedPower=off  ActivePower=94200000  InductivePower=19000000  CapacitivePower=0  Pabc=[10e3 9e3 11e3]  QLabc=[100 90 110]  QCabc=[100 90 110]  Pabcp=Pa_890  QLabcp=Pp_890  QCabcp=Pn_890  Measurements=None  LoadType=constant PQ
  Load7 : spsThreePhaseSeriesRLCLoadLib/Three-Phase Series RLC Load  LConnTagsString=A|B|C  Configuration=Y (grounded)  NominalVoltage=(132000)*1.00738  Vabc=[1e3 1e3 1e3]  Vabcp=V_890*Vnom1  NominalFrequency=60  UnbalancedPower=off  ActivePower=22800000  InductivePower=10900000  CapacitivePower=0  Pabc=[10e3 9e3 11e3]  QLabc=[100 90 110]  QCabc=[100 90 110]  Pabcp=Pa_890  QLabcp=Pp_890  QCabcp=Pn_890  Measurements=None  LoadType=constant PQ
  Load8 : spsThreePhaseSeriesRLCLoadLib/Three-Phase Series RLC Load  LConnTagsString=A|B|C  Configuration=Y (grounded)  NominalVoltage=(132000)*1.01  Vabc=[1e3 1e3 1e3]  Vabcp=V_890*Vnom1  NominalFrequency=60  UnbalancedPower=off  ActivePower=30000000  InductivePower=30000000  CapacitivePower=0  Pabc=[10e3 9e3 11e3]  QLabc=[100 90 110]  QCabc=[100 90 110]  Pabcp=Pa_890  QLabcp=Pp_890  QCabcp=Pn_890  Measurements=None  LoadType=constant PQ
  Low-Pass Filter (Discrete or Continuous){1,3,6..7} (4 alike) : eeGeneralControl/Low-Pass Filter (Discrete or Continuous)  K=1  T=0.01  B=inf  A=-inf  init_option=Inherited from block input  x0=0  Ts=-1
  MultiStateImage : MultiStateImageBlock  LabelPosition=Bottom
  Mux{,1..3} (4 alike) : Mux  Inputs=2
  Mux4 : Mux  Inputs=3
  Mux5 : Mux  Inputs=3
  PWM Generator (2-Level)1 : spsPWMGenerator2LevelLib/PWM Generator (2-Level)  ModulatorType=Three-phase bridge (6 pulses)  ModulatorMode=Unsynchronized  Fc=fsw  Pc=90  nF=27  MinMax="[ -1  1 ]"  SamplingTechnique=Natural  ModulatingSignals=off  m=0.8  Freq=60  Phase=0  Ts=Tss  ShowCarrierOutport=on
  PWM Generator (2-Level)2 : spsPWMGenerator2LevelLib/PWM Generator (2-Level)  ModulatorType=Three-phase bridge (6 pulses)  ModulatorMode=Unsynchronized  Fc=fsw2  Pc=90  nF=27  MinMax="[ -1  1 ]"  SamplingTechnique=Natural  ModulatingSignals=off  m=0.8  Freq=60  Phase=0  Ts=Tss  ShowCarrierOutport=on
  Power Measurement (Three-Phase)1 : eePowerMeasurement/Power Measurement (Three-Phase)  LabelModeActiveChoice=Discrete  F=60  K=[1]  Seq=Positive  Ts=Tss
      settings: SourceProductBaseCode=PS
  Power Measurement (Three-Phase)3 : eePowerMeasurement/Power Measurement (Three-Phase)  LabelModeActiveChoice=Discrete  F=60  K=[1]  Seq=Positive  Ts=Tss
      settings: SourceProductBaseCode=PS
  Power-Flow : Subsystem
      mask Display: disp('Power-Flow\nResults')
  Product1 : Product
  Rbrk1 : spsSeriesRLCBranchLib/Series RLC Branch  LConnTagsString=__new0  RConnTagsString=__new0  BranchType=R  Resistance=Rbrk  Inductance=0.01  SetiL0=off  InitialCurrent=0  Capacitance=C_dc  Setx0=off  InitialVoltage=0  Measurements=None
  Rd : spsSeriesRLCBranchLib/Series RLC Branch  LConnTagsString=__new0  RConnTagsString=__new0  BranchType=R  Resistance=1  Inductance=0.01  SetiL0=off  InitialCurrent=0  Capacitance=C_dc  Setx0=off  InitialVoltage=0  Measurements=None
  Rectifier Control : Subsystem
  Reusens : spsThreePhaseVIMeasurementLib/Three-Phase V-I Measurement  VoltageMeasurement=phase-to-ground  SetLabelV=on  LabelV=Vabc_8  Vpu=on  VpuLL=off  CurrentMeasurement=yes  SetLabelI=on  LabelI=Iabc_8  Ipu=on  Pbase=100e6  Vbase=132e3  OutputType=Magnitude-Angle  PhasorSimulation=off  PSBequivalent=0
  Roanoke : spsThreePhaseVIMeasurementLib/Three-Phase V-I Measurement  VoltageMeasurement=phase-to-ground  SetLabelV=on  LabelV=Vabc_6  Vpu=on  VpuLL=off  CurrentMeasurement=yes  SetLabelI=on  LabelI=Iabc_6  Ipu=on  Pbase=100e6  Vbase=132e3  OutputType=Magnitude-Angle  PhasorSimulation=off  PSBequivalent=0
  Roanoke1 : spsThreePhaseVIMeasurementLib/Three-Phase V-I Measurement  VoltageMeasurement=phase-to-ground  SetLabelV=on  LabelV=Vabc_9  Vpu=on  VpuLL=off  CurrentMeasurement=yes  SetLabelI=on  LabelI=Iabc_9  Ipu=on  Pbase=100e6  Vbase=33e3  OutputType=Magnitude-Angle  PhasorSimulation=off  PSBequivalent=0
  Roanoke2 : spsThreePhaseVIMeasurementLib/Three-Phase V-I Measurement  VoltageMeasurement=phase-to-ground  SetLabelV=on  LabelV=Vabc_10  Vpu=on  VpuLL=off  CurrentMeasurement=yes  SetLabelI=on  LabelI=Iabc_10  Ipu=on  Pbase=100e6  Vbase=33e3  OutputType=Magnitude-Angle  PhasorSimulation=off  PSBequivalent=0
  Roanoke3 : spsThreePhaseVIMeasurementLib/Three-Phase V-I Measurement  VoltageMeasurement=phase-to-ground  SetLabelV=on  LabelV=Vabc_11  Vpu=on  VpuLL=off  CurrentMeasurement=yes  SetLabelI=on  LabelI=Iabc_11  Ipu=on  Pbase=100e6  Vbase=33e3  OutputType=Magnitude-Angle  PhasorSimulation=off  PSBequivalent=0
  Scope : Scope  NumInputPorts=2
  Scope1 : Scope  NumInputPorts=4
  Scope2 : Scope  NumInputPorts=2
  Scope22 : Scope  NumInputPorts=3
  Scope23 : Scope  Commented=on
  Scope24 : Scope
  Scope25 : Scope
  Scope26 : Scope
  Scope27 : Scope  Commented=on
  Scope29 : Scope  Commented=on
  Scope33 : Scope  NumInputPorts=4
  Scope34 : Scope  NumInputPorts=4
  Scope35 : Scope  Commented=on  NumInputPorts=3
  Scope36 : Scope  Commented=on  NumInputPorts=3
  Series RLC Branch1 : spsSeriesRLCBranchLib/Series RLC Branch  LConnTagsString=__new0  RConnTagsString=__new0  BranchType=RL  Resistance=R1  Inductance=L1  SetiL0=off  InitialCurrent=0  Capacitance=Cf1  Setx0=off  InitialVoltage=0  Measurements=None
  Series RLC Branch12 : spsSeriesRLCBranchLib/Series RLC Branch  LConnTagsString=__new0  RConnTagsString=__new0  BranchType=RL  Resistance=R2  Inductance=L2  SetiL0=off  InitialCurrent=0  Capacitance=Cf1  Setx0=off  InitialVoltage=0  Measurements=None
  Series RLC Branch{2..4,7,9,13} (6 alike) : spsSeriesRLCBranchLib/Series RLC Branch  LConnTagsString=__new0  RConnTagsString=__new0  BranchType=R  Resistance=100e3  Inductance=1e-3  SetiL0=off  InitialCurrent=0  Capacitance=Cf1  Setx0=off  InitialVoltage=0  Measurements=None
  Series RLC Branch14 : spsSeriesRLCBranchLib/Series RLC Branch  LConnTagsString=__new0  RConnTagsString=__new0  BranchType=RL  Resistance=R1  Inductance=L1  SetiL0=off  InitialCurrent=0  Capacitance=Cf1  Setx0=off  InitialVoltage=0  Measurements=None
  Series RLC Branch15 : spsSeriesRLCBranchLib/Series RLC Branch  LConnTagsString=__new0  RConnTagsString=__new0  BranchType=RC  Resistance=R_dump  Inductance=0.01  SetiL0=off  InitialCurrent=0  Capacitance=Cf1  Setx0=off  InitialVoltage=0  Measurements=None
  Series RLC Branch16 : spsSeriesRLCBranchLib/Series RLC Branch  LConnTagsString=__new0  RConnTagsString=__new0  BranchType=RC  Resistance=R_dump  Inductance=0.01  SetiL0=off  InitialCurrent=0  Capacitance=Cf1  Setx0=off  InitialVoltage=0  Measurements=None
  Series RLC Branch19 : spsSeriesRLCBranchLib/Series RLC Branch  LConnTagsString=__new0  RConnTagsString=__new0  BranchType=RC  Resistance=R_dump  Inductance=0.01  SetiL0=off  InitialCurrent=0  Capacitance=Cf1  Setx0=off  InitialVoltage=0  Measurements=None
  Series RLC Branch20 : spsSeriesRLCBranchLib/Series RLC Branch  LConnTagsString=__new0  RConnTagsString=__new0  BranchType=RC  Resistance=R_dump2  Inductance=0.01  SetiL0=off  InitialCurrent=0  Capacitance=Cf2  Setx0=off  InitialVoltage=0  Measurements=None
  Series RLC Branch21 : spsSeriesRLCBranchLib/Series RLC Branch  LConnTagsString=__new0  RConnTagsString=__new0  BranchType=RC  Resistance=R_dump2  Inductance=0.01  SetiL0=off  InitialCurrent=0  Capacitance=Cf2  Setx0=off  InitialVoltage=0  Measurements=None
  Series RLC Branch22 : spsSeriesRLCBranchLib/Series RLC Branch  LConnTagsString=__new0  RConnTagsString=__new0  BranchType=RC  Resistance=R_dump2  Inductance=0.01  SetiL0=off  InitialCurrent=0  Capacitance=Cf2  Setx0=off  InitialVoltage=0  Measurements=None
  Series RLC Branch25 : spsSeriesRLCBranchLib/Series RLC Branch  LConnTagsString=__new0  RConnTagsString=__new0  BranchType=C  Resistance=R_dump  Inductance=0.01  SetiL0=off  InitialCurrent=0  Capacitance=C_dc  Setx0=off  InitialVoltage=0  Measurements=None
  Series RLC Branch26 : spsSeriesRLCBranchLib/Series RLC Branch  LConnTagsString=__new0  RConnTagsString=__new0  BranchType=RL  Resistance=Rg2  Inductance=Lg2  SetiL0=off  InitialCurrent=0  Capacitance=Cf2  Setx0=off  InitialVoltage=0  Measurements=None
  Series RLC Branch45 : spsSeriesRLCBranchLib/Series RLC Branch  LConnTagsString=__new0  RConnTagsString=__new0  BranchType=RL  Resistance=Rg2  Inductance=Lg2  SetiL0=off  InitialCurrent=0  Capacitance=Cf2  Setx0=off  InitialVoltage=0  Measurements=None
  Series RLC Branch46 : spsSeriesRLCBranchLib/Series RLC Branch  LConnTagsString=__new0  RConnTagsString=__new0  BranchType=RL  Resistance=Rg2  Inductance=Lg2  SetiL0=off  InitialCurrent=0  Capacitance=Cf2  Setx0=off  InitialVoltage=0  Measurements=None
  Series RLC Branch47 : spsSeriesRLCBranchLib/Series RLC Branch  LConnTagsString=__new0  RConnTagsString=__new0  BranchType=RL  Resistance=Rg1  Inductance=Lg1  SetiL0=off  InitialCurrent=0  Capacitance=Cf1  Setx0=off  InitialVoltage=0  Measurements=None
  Series RLC Branch48 : spsSeriesRLCBranchLib/Series RLC Branch  LConnTagsString=__new0  RConnTagsString=__new0  BranchType=RL  Resistance=Rg1  Inductance=Lg1  SetiL0=off  InitialCurrent=0  Capacitance=Cf1  Setx0=off  InitialVoltage=0  Measurements=None
  Series RLC Branch49 : spsSeriesRLCBranchLib/Series RLC Branch  LConnTagsString=__new0  RConnTagsString=__new0  BranchType=RL  Resistance=Rg1  Inductance=Lg1  SetiL0=off  InitialCurrent=0  Capacitance=Cf1  Setx0=off  InitialVoltage=0  Measurements=None
  Series RLC Branch5 : spsSeriesRLCBranchLib/Series RLC Branch  LConnTagsString=__new0  RConnTagsString=__new0  BranchType=RL  Resistance=R2  Inductance=L2  SetiL0=off  InitialCurrent=0  Capacitance=Cf1  Setx0=off  InitialVoltage=0  Measurements=None
  Series RLC Branch50 : spsSeriesRLCBranchLib/Series RLC Branch  LConnTagsString=__new0  RConnTagsString=__new0  BranchType=RL  Resistance=R1  Inductance=L1  SetiL0=off  InitialCurrent=0  Capacitance=Cf1  Setx0=off  InitialVoltage=0  Measurements=None
  Series RLC Branch6 : spsSeriesRLCBranchLib/Series RLC Branch  LConnTagsString=__new0  RConnTagsString=__new0  BranchType=RL  Resistance=R2  Inductance=L2  SetiL0=off  InitialCurrent=0  Capacitance=Cf1  Setx0=off  InitialVoltage=0  Measurements=None
  Step : Step  Commented=on  Time=5  Before=5e6  After=20e6  SampleTime=0
  Three-Phase V-I Measurement3 : spsThreePhaseVIMeasurementLib/Three-Phase V-I Measurement  VoltageMeasurement=phase-to-ground  SetLabelV=off  LabelV=Vabc  Vpu=off  VpuLL=off  CurrentMeasurement=yes  SetLabelI=off  LabelI=Iabc  Ipu=off  Pbase=100e6  Vbase=33e3  OutputType=Complex  PhasorSimulation=off  PSBequivalent=0
  Three-Phase V-I Measurement4 : spsThreePhaseVIMeasurementLib/Three-Phase V-I Measurement  VoltageMeasurement=phase-to-ground  SetLabelV=off  LabelV=Vabc  Vpu=off  VpuLL=off  CurrentMeasurement=yes  SetLabelI=off  LabelI=Iabc  Ipu=off  Pbase=100e6  Vbase=33e3  OutputType=Complex  PhasorSimulation=off  PSBequivalent=0
  To Workspace5 : ToWorkspace  VariableName=Vabc  SaveFormat=Timeseries  SampleTime=-1
  To Workspace6 : ToWorkspace  VariableName=Iabc  SaveFormat=Timeseries  SampleTime=-1
  To Workspace7 : ToWorkspace  VariableName=Vabc3  SaveFormat=Timeseries  SampleTime=-1
  To Workspace8 : ToWorkspace  VariableName=Iabc3  SaveFormat=Timeseries  SampleTime=-1
  Transformer1 132kV / 33kV2 : spsThreePhaseTransformerTwoWindingsLib/Three-Phase Transformer (Two Windings)  Winding1Connection=Yg  Winding2Connection=Yg  CoreType=Three single-phase transformers  SetSaturation=off  Hysteresis=off  DataFile='hysteresis'  SetInitialFlux=off  Measurements=None  UNITS=pu  NominalPower=[100e6, 60]  Winding1=[132e3, 0, 6.7906e-4]  Winding2=[33e3, 0, 6.7906e-4]  Rm=2000  Lm=1000  L0=0.5  Saturation=[ 0,0 ; 0.0024,1.2 ; 1.0,1.52 ]  InitialFluxes=[ 0.8 , -0.8 , 0.7 ]  BreakLoop=off  DiscreteSolver=Trapezoidal iterative  DataType=off  TransfoNumber=1
  Transformer2 132kV / 33kV : spsThreePhaseTransformerTwoWindingsLib/Three-Phase Transformer (Two Windings)  Winding1Connection=Yg  Winding2Connection=Yg  CoreType=Three single-phase transformers  SetSaturation=off  Hysteresis=off  DataFile='hysteresis'  SetInitialFlux=off  Measurements=None  UNITS=pu  NominalPower=[100e6, 60]  Winding1=[132e3, 0, 5.5174e-4]  Winding2=[33e3, 0, 5.5174e-4]  Rm=2000  Lm=1000  L0=0.5  Saturation=[ 0,0 ; 0.0024,1.2 ; 1.0,1.52 ]  InitialFluxes=[ 0.8 , -0.8 , 0.7 ]  BreakLoop=off  DiscreteSolver=Trapezoidal iterative  DataType=off  TransfoNumber=1
  Transformer3 132kV / 33kV : spsThreePhaseTransformerTwoWindingsLib/Three-Phase Transformer (Two Windings)  Winding1Connection=Yg  Winding2Connection=Yg  CoreType=Three single-phase transformers  SetSaturation=off  Hysteresis=off  DataFile='hysteresis'  SetInitialFlux=off  Measurements=None  UNITS=pu  NominalPower=[ 100e6 , 60 ]  Winding1=[ 132e3 , 0 , 1.4748e-3 ]  Winding2=[ 33e3 , 0 , 1.4748e-3 ]  Rm=2000  Lm=1000  L0=0.5  Saturation=[ 0,0 ; 0.0024,1.2 ; 1.0,1.52 ]  InitialFluxes=[ 0.8 , -0.8 , 0.7 ]  BreakLoop=off  DiscreteSolver=Trapezoidal iterative  DataType=off  TransfoNumber=1
  Transformer4 132kV / 33kV : spsThreePhaseTransformerTwoWindingsLib/Three-Phase Transformer (Two Windings)  Winding1Connection=Yg  Winding2Connection=Yg  CoreType=Three single-phase transformers  SetSaturation=off  Hysteresis=off  DataFile='hysteresis'  SetInitialFlux=off  Measurements=None  UNITS=pu  NominalPower=[ 100e6 , 60 ]  Winding1=[ 132e3 , 0 , 1.0504e-3 ]  Winding2=[ 33e3 , 0 , 1.0504e-3 ]  Rm=2000  Lm=1000  L0=0.5  Saturation=[ 0,0 ; 0.0024,1.2 ; 1.0,1.52 ]  InitialFluxes=[ 0.8 , -0.8 , 0.7 ]  BreakLoop=off  DiscreteSolver=Trapezoidal iterative  DataType=off  TransfoNumber=1
  Universal Bridge1 : spsUniversalBridgeLib/Universal Bridge  Arms=3  SnubberResistance=1e6  SnubberCapacitance=inf  Device=IGBT / Diodes  Ron=1e-6  Lon=0  ForwardVoltages="[  0  0  ]"  ForwardVoltage=0  GTOparameters=[ 10e-6 , 20e-6 ]  IGBTparameters=[ 1e-6 , 2e-6 ]  Measurements=None  Measurements_2=None  converterType=Rectifier
  Universal Bridge2 : spsUniversalBridgeLib/Universal Bridge  Arms=3  SnubberResistance=1e6  SnubberCapacitance=inf  Device=IGBT / Diodes  Ron=1e-6  Lon=0  ForwardVoltages="[  0  0  ]"  ForwardVoltage=0  GTOparameters=[ 10e-6 , 20e-6 ]  IGBTparameters=[ 1e-6 , 2e-6 ]  Measurements=None  Measurements_2=None  converterType=Rectifier
  Va1 : spsVoltageMeasurementLib/Voltage Measurement  PhasorSimulation=off  OutputType=Complex  PSBequivalent=0
  Va2 : spsVoltageMeasurementLib/Voltage Measurement  PhasorSimulation=off  OutputType=Complex  PSBequivalent=0
  Vb1 : spsVoltageMeasurementLib/Voltage Measurement  PhasorSimulation=off  OutputType=Complex  PSBequivalent=0
  Vb2 : spsVoltageMeasurementLib/Voltage Measurement  PhasorSimulation=off  OutputType=Complex  PSBequivalent=0
  Vc1 : spsVoltageMeasurementLib/Voltage Measurement  PhasorSimulation=off  OutputType=Complex  PSBequivalent=0
  Vc2 : spsVoltageMeasurementLib/Voltage Measurement  PhasorSimulation=off  OutputType=Complex  PSBequivalent=0
  Vdc_meas2 : spsVoltageMeasurementLib/Voltage Measurement  PhasorSimulation=off  OutputType=Complex  PSBequivalent=0
  Vmeas1 : spsVoltageMeasurementLib/Voltage Measurement  PhasorSimulation=off  OutputType=Complex  PSBequivalent=0
  Voltage Measurement{1..9} (9 alike) : spsVoltageMeasurementLib/Voltage Measurement  PhasorSimulation=off  OutputType=Complex  PSBequivalent=0
  powergui : spspowerguiLib/powergui  Priority=1  SimulationMode=Discrete  SampleTime=Tss  frequency=60  Iterations=50  frequencyindice=60  Pbase=100e3  ErrMax=0.0001  UnitsV=kV  UnitsW=kW  buscounter=0  FunctionMessages=off  echomessages=off  EnableUseOfTLC=off  CurrentSourceSwitches=off  DisableSnubberDevices=off  DisableRonSwitches=off  DisableVfSwitches=off  DisplayEquations=off  AutomaticDiscreteSolvers=off  SolverType=Tustin/Backward Euler (TBE)  Interpol=off  ExternalGateDelay=off  methode=off  Ts=100  x0status=blocks  SPID=off  SwTol=0  HookPort=off  NonlinearTolerance=1e-4  nMaxIteration=100  ContinueOnMaxIteration=off  RestoreLinks=warning  ResistiveCurrentMeasurement=off  Frange=[0:2:500]  Ylog=off  Xlog=on  ShowGrid=off  save=off  variable=ZData  structure=logsout  ZoomFFT=on  StartTime=0.0  cycles=1  DisplayStyle=1  fundamental=60  FreqAxis=off  MaxFrequency=1000  frequencyindicesteady=1  RmsSteady=1  display=off
  shunt 10 : spsThreePhaseSeriesRLCLoadLib/Three-Phase Series RLC Load  LConnTagsString=A|B|C  Configuration=Y (grounded)  NominalVoltage=33e3  Vabc=[1e3 1e3 1e3]  Vabcp=V_890*Vnom1  NominalFrequency=60  UnbalancedPower=off  ActivePower=0  InductivePower=0  CapacitivePower=19000000  Pabc=[10e3 9e3 11e3]  QLabc=[100 90 110]  QCabc=[100 90 110]  Pabcp=Pa_890  QLabcp=Pp_890  QCabcp=Pn_890  Measurements=None  LoadType=constant Z
  shunt 24 : spsThreePhaseSeriesRLCLoadLib/Three-Phase Series RLC Load  LConnTagsString=A|B|C  Configuration=Y (grounded)  NominalVoltage=33e3  Vabc=[1e3 1e3 1e3]  Vabcp=V_890*Vnom1  NominalFrequency=60  UnbalancedPower=off  ActivePower=0  InductivePower=0  CapacitivePower=4300000  Pabc=[10e3 9e3 11e3]  QLabc=[100 90 110]  QCabc=[100 90 110]  Pabcp=Pa_890  QLabcp=Pp_890  QCabcp=Pn_890  Measurements=None  LoadType=constant Z
  tag scope: Vdc_measure=global, pulse1=global, pulse2=global
  wires:
  Voltage Measurement4/1 -> [Vbc1]
  Low-Pass Filter (Discrete or Continuous)6/1 -> Mux2/2, Display7/1  "Real power [W]"
  Constant3/1 -> Rectifier Control/7(P_ref)
  Current Measurement8/1 -> Rectifier Control/4(Ia)
  Current Measurement1/1 -> [Iga1_rms]
  Voltage Measurement3/1 -> [Vab1]
  Step/1 -> Scope23/1
  Voltage Measurement5/1 -> [Vdc_measure]
  [Vdc_measure] -> Display1/1, Scope22/1, Product1/1
  Voltage Measurement9/1 -> [Vbc2]
  [Iga1_rms] -> Scope33/2
  Vdc_meas2/1 -> Break control1/1(Vdc)
  Va1/1 -> Scope35/1, Rectifier Control/1(Va)
  Current Measurement9/1 -> Rectifier Control/5(Ib)
  Constant4/1 -> Rectifier Control/8(Q_ref)
  [Ivsc_a2_rms] -> Scope34/4
  Three-Phase V-I Measurement4/2 -> Scope27/1, Power Measurement (Three-Phase)3/2, To Workspace8/1
  Low-Pass Filter (Discrete or Continuous)1/1 -> Display14/1, Mux/2  "Real power [W]"
  Current Measurement13/1 -> [Igb2_rms]
  Power Measurement (Three-Phase)1/2 -> Mux1/2, Display15/1, Low-Pass Filter (Discrete or Continuous)3/1
  Voltage Measurement6/1 -> [Vab2_rms]
  Vmeas1/1 -> Inverter Control/7(Vdc_link)
  Current Measurement2/1 -> [Igc2_rms]
  Vc2/1 -> Inverter Control/3(Vc), Scope36/3
  Power Measurement (Three-Phase)3/2 -> Mux3/2, Display8/1, Low-Pass Filter (Discrete or Continuous)7/1
  Va2/1 -> Scope36/1, Inverter Control/1(Va)
  PWM Generator (2-Level)1/1 -> Mux4/2, [pulse1]
  [Vab2] -> Scope34/3
  Power Measurement (Three-Phase)3/1 -> Mux2/1, Display18/1, Low-Pass Filter (Discrete or Continuous)6/1
  Low-Pass Filter (Discrete or Continuous)3/1 -> Mux1/1, Display16/1  "Reactive power [var]"
  Product1/1 -> Display17/1, Scope22/2
  Three-Phase V-I Measurement3/2 -> Scope25/1, Power Measurement (Three-Phase)1/2, To Workspace6/1
  Low-Pass Filter (Discrete or Continuous)7/1 -> Display13/1, Mux3/1  "Reactive power [var]"
  Current Measurement7/1 -> [Igc1_rms]
  Current Measurement12/1 -> [Iga2_rms]
  [Vabc1] -> Mux4/1, PWM Generator (2-Level)1/1
  Current Measurement10/1 -> Rectifier Control/6(Ic)
  Current Measurement5/1 -> Inverter Control/6(Ic)
  [pulse1] -> Universal Bridge2/1
  Break control1/1(S_break) -> Scope29/1, Breaker1/1
  [Vabc2] -> Mux5/1, PWM Generator (2-Level)2/1
  PWM Generator (2-Level)2/1 -> Mux5/2, [pulse2]
  Vc1/1 -> Scope35/3, Rectifier Control/3(Vc)
  Three-Phase V-I Measurement3/1 -> Scope24/1, Power Measurement (Three-Phase)1/1, To Workspace5/1
  [Vab1] -> Scope33/3
  Voltage Measurement7/1 -> [Vbc2_rms]
  Power Measurement (Three-Phase)1/1 -> Mux/1, Display6/1, Low-Pass Filter (Discrete or Continuous)1/1
  [Idc_link] -> Product1/2, Display2/1, Scope22/3
  Voltage Measurement2/1 -> [Vbc1_rms]
  Three-Phase V-I Measurement4/1 -> Scope26/1, Power Measurement (Three-Phase)3/1, To Workspace7/1
  Current Measurement6/1 -> [Igb1_rms]
  Current Measurement4/1 -> Inverter Control/5(Ib)
  Voltage Measurement8/1 -> [Vab2]
  Vb1/1 -> Rectifier Control/2(Vb), Scope35/2
  [pulse2] -> Universal Bridge1/1
  Current Measurement3/1 -> Inverter Control/4(Ia)
  Current Measurement11/1 -> [Idc_link]
  Voltage Measurement1/1 -> [Vab1_rms]
  [Iga2_rms] -> Scope34/2
  Vb2/1 -> Scope36/2, Inverter Control/2(Vb)
  [Ivsc_a1_rms] -> Scope33/4
  Mux/1 -> Scope/1
  Mux1/1 -> Scope/2
  Mux2/1 -> Scope2/1
  Mux3/1 -> Scope2/2
  PWM Generator (2-Level)1/2 -> Mux4/3
  PWM Generator (2-Level)2/2 -> Mux5/3
  Mux4/1 -> Scope1/2
  Mux5/1 -> Scope1/3
  [Vab1] -> Scope1/1
  [Vdc_measure] -> Scope1/4
  Current Measurement14/1 -> [Ivsc_a1_rms]
  [Vab1_rms] -> Scope33/1
  [Vab2_rms] -> Scope34/1
  Current Measurement15/1 -> [Ivsc_a2_rms]
  connections:
  Series RLC Branch20/RConn1 -- Series RLC Branch21/RConn1 -- Series RLC Branch22/RConn1
  Universal Bridge2/LConn1 -- Voltage Measurement3/LConn1 -- Current Measurement14/RConn1
  Current Measurement7/RConn1 -- Current Measurement10/LConn1 -- Voltage Measurement2/LConn2 -- Series RLC Branch4/RConn1 -- Vc1/LConn1 -- Series RLC Branch19/LConn1
  Voltage Measurement5/LConn2 -- Universal Bridge2/RConn2 -- Vmeas1/LConn2 -- Universal Bridge1/RConn2 -- Rbrk1/RConn1 -- Vdc_meas2/LConn2 -- Series RLC Branch25/RConn1
  Series RLC Branch15/RConn1 -- Series RLC Branch16/RConn1 -- Series RLC Branch19/RConn1
  Current Measurement1/RConn1 -- Va1/LConn1 -- Series RLC Branch2/RConn1 -- Current Measurement8/LConn1 -- Voltage Measurement1/LConn1 -- Series RLC Branch15/LConn1
  Series RLC Branch13/RConn1 -- Vc2/LConn1 -- Series RLC Branch6/LConn1 -- Voltage Measurement7/LConn2 -- Current Measurement2/RConn1 -- Series RLC Branch20/LConn1
  Voltage Measurement2/LConn1 -- Current Measurement9/LConn1 -- Vb1/LConn1 -- Series RLC Branch3/RConn1 -- Series RLC Branch16/LConn1 -- Current Measurement6/RConn1 -- Voltage Measurement1/LConn2
  Series RLC Branch1/RConn1 -- Voltage Measurement4/LConn2 -- Universal Bridge2/LConn3
  Voltage Measurement9/LConn1 -- Voltage Measurement8/LConn2 -- Current Measurement4/RConn1 -- Universal Bridge1/LConn2
  Va1/LConn2 -- Series RLC Branch4/LConn1 -- Vc1/LConn2 -- Vb1/LConn2 -- Series RLC Branch3/LConn1 -- Series RLC Branch2/LConn1
  Current Measurement13/RConn1 -- Series RLC Branch21/LConn1 -- Voltage Measurement6/LConn2 -- Series RLC Branch5/LConn1 -- Voltage Measurement7/LConn1 -- Series RLC Branch9/RConn1 -- Vb2/LConn1
  Voltage Measurement9/LConn2 -- Universal Bridge1/LConn3 -- Current Measurement5/RConn1
  Series RLC Branch12/LConn1 -- Series RLC Branch7/RConn1 -- Va2/LConn1 -- Series RLC Branch22/LConn1 -- Current Measurement12/RConn1 -- Voltage Measurement6/LConn1
  Universal Bridge1/LConn1 -- Current Measurement15/RConn1 -- Voltage Measurement8/LConn1
  Vdc_meas2/LConn1 -- Universal Bridge1/RConn1 -- Vmeas1/LConn1 -- Breaker1/RConn1 -- Series RLC Branch25/LConn1 -- Rd/RConn1
  Universal Bridge2/LConn2 -- Voltage Measurement4/LConn1 -- Voltage Measurement3/LConn2 -- Series RLC Branch50/RConn1
  Series RLC Branch9/LConn1 -- Vc2/LConn2 -- Series RLC Branch13/LConn1 -- Vb2/LConn2 -- Series RLC Branch7/LConn1 -- Va2/LConn2
  Current Measurement8/RConn1 -- Series RLC Branch14/LConn1
  Series RLC Branch45/RConn1 -- Current Measurement13/LConn1
  Three-Phase V-I Measurement3/RConn2 -- Series RLC Branch48/LConn1
  Series RLC Branch46/LConn1 -- Three-Phase V-I Measurement4/RConn3
  Transformer1 132kV / 33kV2/RConn3 -- Three-Phase V-I Measurement3/LConn3
  Series RLC Branch26/LConn1 -- Three-Phase V-I Measurement4/RConn1
  Series RLC Branch6/RConn1 -- Current Measurement5/LConn1
  Series RLC Branch12/RConn1 -- Current Measurement3/LConn1
  Series RLC Branch45/LConn1 -- Three-Phase V-I Measurement4/RConn2
  Series RLC Branch5/RConn1 -- Current Measurement4/LConn1
  Series RLC Branch26/RConn1 -- Current Measurement12/LConn1
  Series RLC Branch47/RConn1 -- Current Measurement1/LConn1
  Three-Phase V-I Measurement3/RConn3 -- Series RLC Branch49/LConn1
  Series RLC Branch49/RConn1 -- Current Measurement7/LConn1
  Rbrk1/LConn1 -- Breaker1/LConn1
  Transformer1 132kV / 33kV2/RConn1 -- Three-Phase V-I Measurement3/LConn1
  Current Measurement9/RConn1 -- Series RLC Branch50/LConn1
  Universal Bridge2/RConn1 -- Current Measurement11/LConn1
  Series RLC Branch48/RConn1 -- Current Measurement6/LConn1
  Transformer1 132kV / 33kV2/RConn2 -- Three-Phase V-I Measurement3/LConn2
  Series RLC Branch46/RConn1 -- Current Measurement2/LConn1
  Three-Phase V-I Measurement3/RConn1 -- Series RLC Branch47/LConn1
  Current Measurement10/RConn1 -- Series RLC Branch1/LConn1
  Rd/LConn1 -- Current Measurement11/RConn1 -- Voltage Measurement5/LConn1
  L2-6/RConn2 -- L6-8/LConn2 -- L4-6/RConn2 -- Roanoke/RConn2 -- L6-7/RConn2
  L6-7/RConn1 -- Roanoke/RConn1 -- L4-6/RConn1 -- Load Flow Bus43/LConn1 -- L6-8/LConn1 -- L2-6/RConn1
  24/RConn3 -- L23-24/RConn3 -- L22-24/LConn3 -- L24-25/LConn3
  L12-16/LConn1 -- L12-15/LConn1 -- L12-14/LConn1 -- Load Flow Bus57/LConn1 -- Hancock1/RConn1 -- L12-13/RConn1 -- Three-Phase V-I Measurement4/LConn1
  L6-7/LConn1 -- Load Flow Bus42/LConn1 -- Blaine/LConn1 -- L5-7/RConn1
  Cloverdl1/RConn1 -- L6-28/RConn1 -- L8-28/RConn1
  23/LConn2 -- L23-24/LConn2 -- L15-23/RConn2
  L1-3/LConn3 -- Glen Lyn/LConn3 -- L1-2/RConn3
  L3-4/RConn2 -- Transformer1 132kV / 33kV2/LConn2 -- L2-4/RConn2 -- L4-6/LConn2 -- Hancock/RConn2
  L22-24/LConn1 -- L23-24/RConn1 -- 24/RConn1 -- L24-25/LConn1
  Load Flow Bus5/LConn1 -- 14/RConn1 -- L12-14/RConn1 -- L14-15/LConn1
  15/LConn1 -- L15-18/LConn1 -- L14-15/RConn1 -- L12-15/RConn1 -- L15-23/LConn1 -- Load Flow Bus64/LConn1
  Load Flow Bus8/LConn1 -- L25-26/RConn1 -- 26/RConn1
  Fieldale/LConn1 -- Load Flow Bus1/LConn1 -- L2-5/RConn1 -- L5-7/LConn1
  L23-24/LConn3 -- 23/LConn3 -- L15-23/RConn3
  shunt 24/LConn1 -- Load24/LConn1 -- Load Flow Bus9/LConn1 -- 24/LConn1
  Hancock/RConn1 -- L2-4/RConn1 -- L4-6/LConn1 -- Transformer1 132kV / 33kV2/LConn1 -- L3-4/RConn1 -- Load Flow Bus3/LConn1
  L12-14/LConn2 -- L12-15/LConn2 -- L12-16/LConn2 -- Three-Phase V-I Measurement4/LConn2 -- L12-13/RConn2 -- Hancock1/RConn2
  Transformer2 132kV / 33kV/LConn2 -- Transformer3 132kV / 33kV/LConn2 -- L6-28/LConn2 -- Roanoke/LConn2
  18/RConn2 -- L15-18/RConn2 -- L18-19/LConn2
  25/RConn1 -- L24-25/RConn1 -- L25-26/LConn1
  30/RConn2 -- L27-30/LConn2 -- L29-30/LConn2
  Hancock/RConn3 -- L2-4/RConn3 -- L4-6/LConn3 -- Transformer1 132kV / 33kV2/LConn3 -- L3-4/RConn3
  L10-20/RConn2 -- L10-17/RConn2 -- L9-10/RConn2 -- Roanoke2/RConn2 -- L10-22/LConn2 -- L10-21/LConn2 -- Transformer3 132kV / 33kV/RConn2
  Claytor/RConn3 -- Gen2/RConn3 -- Load2/LConn3
  21/RConn3 -- L10-21/RConn3 -- L21-22/LConn3
  shunt 24/LConn2 -- Load24/LConn2 -- 24/LConn2
  L8-28/LConn3 -- L6-8/RConn3 -- Reusens/RConn3
  Kumis/RConn3 -- L3-4/LConn3 -- L1-3/RConn3
  L12-15/RConn2 -- L14-15/RConn2 -- L15-23/LConn2 -- 15/LConn2 -- L15-18/LConn2
  19/RConn3 -- L18-19/RConn3 -- L19-20/RConn3
  Hancock1/RConn3 -- Three-Phase V-I Measurement4/LConn3 -- L12-16/LConn3 -- L12-13/RConn3 -- L12-14/LConn3 -- L12-15/LConn3
  21/RConn2 -- L10-21/RConn2 -- L21-22/LConn2
  L10-21/RConn1 -- 21/RConn1 -- Load Flow Bus6/LConn1 -- L21-22/LConn1
  L1-2/LConn2 -- Claytor/LConn2 -- L2-4/LConn2 -- L2-6/LConn2 -- L2-5/LConn2
  Gen4/RConn1 -- Reusens/LConn1 -- Load8/LConn1
  Load12/LConn3 -- Hancock1/LConn3 -- Equivalent Gen/RConn3
  16/LConn3 -- L16-17/LConn3 -- L12-16/RConn3
  20/LConn2 -- L10-20/LConn2 -- L19-20/LConn2
  17/LConn3 -- L16-17/RConn3 -- L10-17/LConn3
  L3-4/LConn1 -- Kumis/RConn1 -- Load Flow Bus4/LConn1 -- L1-3/RConn1
  Transformer2 132kV / 33kV/LConn1 -- Roanoke/LConn1 -- L6-28/LConn1 -- Transformer3 132kV / 33kV/LConn1
  L9-11/LConn1 -- Roanoke3/LConn1 -- Load Flow Bus63/LConn1
  L10-17/RConn3 -- Transformer3 132kV / 33kV/RConn3 -- Roanoke2/RConn3 -- L10-22/LConn3 -- L10-21/LConn3 -- L10-20/RConn3 -- L9-10/RConn3
  Transformer2 132kV / 33kV/RConn3 -- L9-10/LConn3 -- Roanoke1/LConn3
  Load Flow Bus28/LConn1 -- Glen Lyn/RConn1 -- Gen1/RConn1
  Reusens/LConn3 -- Gen4/RConn3 -- Load8/LConn3
  Load Flow Bus46/LConn1 -- Cloverdl/RConn1 -- L27-29/RConn1 -- L27-30/RConn1 -- L25-27/RConn1
  Transformer4 132kV / 33kV/LConn1 -- Cloverdl1/LConn1 -- Load Flow Bus45/LConn1
  Fieldale/RConn2 -- Gen3/RConn2 -- Load5/LConn2
  Transformer3 132kV / 33kV/LConn3 -- Transformer2 132kV / 33kV/LConn3 -- Roanoke/LConn3 -- L6-28/LConn3
  Load Flow Bus53/LConn1 -- Roanoke1/LConn1 -- L9-10/LConn1 -- Transformer2 132kV / 33kV/RConn1
  25/LConn1 -- Load Flow Bus10/LConn1 -- L25-27/LConn1
  Fieldale/RConn3 -- Gen3/RConn3 -- Load5/LConn3
  L27-30/RConn3 -- L27-29/RConn3 -- Cloverdl/RConn3 -- L25-27/RConn3
  shunt 10/LConn1 -- Load10/LConn1 -- Roanoke2/LConn1
  Load Flow Bus62/LConn1 -- 20/LConn1 -- L19-20/LConn1 -- L10-20/LConn1
  Load Flow Bus7/LConn1 -- 19/RConn1 -- L18-19/RConn1 -- L19-20/RConn1
  Roanoke2/LConn3 -- shunt 10/LConn3 -- Load10/LConn3
  Glen Lyn/LConn2 -- L1-3/LConn2 -- L1-2/RConn2
  15/LConn3 -- L14-15/RConn3 -- L12-15/RConn3 -- L15-18/LConn3 -- L15-23/LConn3
  Load Flow Bus37/LConn1 -- Gen2/RConn1 -- Load2/LConn1 -- Claytor/RConn1
  Reusens/LConn2 -- Gen4/RConn2 -- Load8/LConn2
  Glen Lyn/LConn1 -- L1-3/LConn1 -- L1-2/RConn1
  L12-13/LConn1 -- Load Flow Bus58/LConn1 -- Hancock2/LConn1
  Claytor/LConn1 -- L1-2/LConn1 -- L2-4/LConn1 -- L2-5/LConn1 -- L2-6/LConn1
  Hancock1/LConn2 -- Load12/LConn2 -- Equivalent Gen/RConn2
  L8-28/RConn3 -- L6-28/RConn3 -- Cloverdl1/RConn3
  L16-17/RConn1 -- 17/LConn1 -- Load Flow Bus55/LConn1 -- L10-17/LConn1
  Load Flow Bus13/LConn1 -- 22/RConn1 -- L21-22/RConn1 -- L10-22/RConn1
  shunt 10/LConn2 -- Load10/LConn2 -- Roanoke2/LConn2
  22/RConn2 -- L10-22/RConn2 -- L21-22/RConn2
  Load Flow Bus12/LConn1 -- 30/RConn1 -- L29-30/LConn1 -- L27-30/LConn1
  L16-17/LConn1 -- 16/LConn1 -- Load Flow Bus56/LConn1 -- L12-16/RConn1
  L8-28/LConn2 -- L6-8/RConn2 -- Reusens/RConn2
  Load Flow Bus11/LConn1 -- 29/RConn1 -- L29-30/RConn1 -- L27-29/LConn1
  29/RConn3 -- L27-29/LConn3 -- L29-30/RConn3
  L4-6/RConn3 -- Roanoke/RConn3 -- L6-8/LConn3 -- L6-7/RConn3 -- L2-6/RConn3
  shunt 24/LConn3 -- Load24/LConn3 -- 24/LConn3
  22/RConn3 -- L10-22/RConn3 -- L21-22/RConn3
  Cloverdl1/RConn2 -- L6-28/RConn2 -- L8-28/RConn2
  L10-22/LConn1 -- Roanoke2/RConn1 -- Load Flow Bus54/LConn1 -- L9-10/RConn1 -- L10-17/RConn1 -- L10-20/RConn1 -- Transformer3 132kV / 33kV/RConn1 -- L10-21/LConn1
  19/RConn2 -- L18-19/RConn2 -- L19-20/RConn2
  L2-4/LConn3 -- L2-5/LConn3 -- L2-6/LConn3 -- L1-2/LConn3 -- Claytor/LConn3
  25/RConn2 -- L24-25/RConn2 -- L25-26/LConn2
  Fieldale/LConn3 -- L5-7/LConn3 -- L2-5/RConn3
  Fieldale/RConn1 -- Gen3/RConn1 -- Load5/LConn1
  L5-7/RConn2 -- L6-7/LConn2 -- Blaine/LConn2
  30/RConn3 -- L29-30/LConn3 -- L27-30/LConn3
  18/RConn3 -- L18-19/LConn3 -- L15-18/RConn3
  Fieldale/LConn2 -- L5-7/LConn2 -- L2-5/RConn2
  29/RConn2 -- L27-29/LConn2 -- L29-30/RConn2
  14/RConn3 -- L14-15/LConn3 -- L12-14/RConn3
  20/LConn3 -- L19-20/LConn3 -- L10-20/LConn3
  L27-30/RConn2 -- Cloverdl/RConn2 -- L25-27/RConn2 -- L27-29/RConn2
  L15-23/RConn1 -- Load Flow Bus52/LConn1 -- 23/LConn1 -- L23-24/LConn1
  16/LConn2 -- L16-17/LConn2 -- L12-16/RConn2
  Claytor/RConn2 -- Gen2/RConn2 -- Load2/LConn2
  L6-7/LConn3 -- L5-7/RConn3 -- Blaine/LConn3
  Reusens/RConn1 -- L6-8/RConn1 -- L8-28/LConn1 -- Load Flow Bus44/LConn1
  17/LConn2 -- L16-17/RConn2 -- L10-17/LConn2
  Load12/LConn1 -- Hancock1/LConn1 -- Equivalent Gen/RConn1
  Load Flow Bus2/LConn1 -- 18/RConn1 -- L15-18/RConn1 -- L18-19/LConn1
  Transformer2 132kV / 33kV/RConn2 -- Roanoke1/LConn2 -- L9-10/LConn2
  24/RConn2 -- L23-24/RConn2 -- L22-24/LConn2 -- L24-25/LConn2
  25/RConn3 -- L24-25/RConn3 -- L25-26/LConn3
  Kumis/RConn2 -- L1-3/RConn2 -- L3-4/LConn2
  14/RConn2 -- L14-15/LConn2 -- L12-14/RConn2
  25/LConn2 -- L25-27/LConn2
  Load3/LConn2 -- Kumis/LConn2
  20/RConn1 -- Load20/LConn1
  Load29/LConn1 -- 29/LConn1
  Load26/LConn3 -- 26/LConn3
  Load15/LConn1 -- 15/RConn1
  Load15/LConn3 -- 15/RConn3
  14/LConn3 -- Load14/LConn3
  Roanoke3/RConn3 -- Gen5/RConn3
  Hancock/LConn3 -- Load4/LConn3
  19/LConn1 -- Load19/LConn1
  22/LConn1 -- L22-24/RConn1
  Load18/LConn1 -- 18/LConn1
  Gen6/RConn3 -- Hancock2/RConn3
  Transformer4 132kV / 33kV/RConn3 -- Cloverdl/LConn3
  19/LConn3 -- Load19/LConn3
  17/RConn3 -- Load17/LConn3
  Load3/LConn1 -- Kumis/LConn1
  Transformer4 132kV / 33kV/LConn3 -- Cloverdl1/LConn3
  Load23/LConn3 -- 23/RConn3
  Load19/LConn2 -- 19/LConn2
  Transformer4 132kV / 33kV/RConn2 -- Cloverdl/LConn2
  Blaine/RConn2 -- Load7/LConn2
  Gen1/RConn3 -- Glen Lyn/RConn3
  Roanoke1/RConn3 -- L9-11/RConn3
  26/RConn2 -- L25-26/RConn2
  16/RConn1 -- Load16/LConn1
  Gen6/RConn2 -- Hancock2/RConn2
  23/RConn2 -- Load23/LConn2
  20/RConn2 -- Load20/LConn2
  30/LConn1 -- Load30/LConn1
  Load29/LConn3 -- 29/LConn3
  Transformer4 132kV / 33kV/RConn1 -- Cloverdl/LConn1
  L9-11/LConn2 -- Roanoke3/LConn2
  17/RConn2 -- Load17/LConn2
  17/RConn1 -- Load17/LConn1
  21/LConn2 -- Load21/LConn2
  Cloverdl1/LConn2 -- Transformer4 132kV / 33kV/LConn2
  Roanoke1/RConn2 -- L9-11/RConn2
  Roanoke3/RConn2 -- Gen5/RConn2
  L9-11/LConn3 -- Roanoke3/LConn3
  Hancock2/LConn3 -- L12-13/LConn3
  Load30/LConn2 -- 30/LConn2
  16/RConn2 -- Load16/LConn2
  20/RConn3 -- Load20/LConn3
  Blaine/RConn1 -- Load7/LConn1
  21/LConn1 -- Load21/LConn1
  22/LConn2 -- L22-24/RConn2
  Load14/LConn2 -- 14/LConn2
  L25-26/RConn3 -- 26/RConn3
  21/LConn3 -- Load21/LConn3
  Hancock/LConn2 -- Load4/LConn2
  Gen1/RConn2 -- Glen Lyn/RConn2
  26/LConn1 -- Load26/LConn1
  Hancock/LConn1 -- Load4/LConn1
  25/LConn3 -- L25-27/LConn3
  Load29/LConn2 -- 29/LConn2
  18/LConn3 -- Load18/LConn3
  Load3/LConn3 -- Kumis/LConn3
  Load30/LConn3 -- 30/LConn3
  L12-13/LConn2 -- Hancock2/LConn2
  Load15/LConn2 -- 15/RConn2
  Hancock2/RConn1 -- Gen6/RConn1
  22/LConn3 -- L22-24/RConn3
  Load18/LConn2 -- 18/LConn2
  23/RConn1 -- Load23/LConn1
  Load14/LConn1 -- 14/LConn1
  26/LConn2 -- Load26/LConn2
  Blaine/RConn3 -- Load7/LConn3
  Roanoke1/RConn1 -- L9-11/RConn1
  Roanoke3/RConn1 -- Gen5/RConn1
  16/RConn3 -- Load16/LConn3
  Current Measurement14/LConn1 -- Series RLC Branch14/RConn1
  Current Measurement3/RConn1 -- Current Measurement15/LConn1
